simulink model "model"  (R2014a)
(part 2 of 3)

  _CN_357523602_330000_CN_87761736_330000 : powerlib/Elements/Distributed Parameters Line  Phases=3  Frequency=60  Resistance=[0.01273 0.3864]  Inductance="[0.9337e-3  4.1264e-3]"  Capacitance=[12.74e-9 7.751e-9]  Length=161.4395  x1=[0 0 0 0; 0.0001244 0 0 0; 0.0002488 0 0 0; 0.0003733 0 0 0; 0.0004977 0 0 0; 0.0006221 0 0 0]  x2=[0 0 0 0; 0.0001244 0 0 0; 0.0002488 0 0 0; 0.0003733 0 0 0; 0.0004977 0 0 0; 0.0006221 0 0 0]  x3=[0 0 0 0; 0.0001244 0 0 0; 0.0002488 0 0 0; 0.0003733 0 0 0; 0.0004977 0 0 0; 0.0006221 0 0 0]  x4=[0 0 0 0; 0.0001244 0 0 0; 0.0002488 0 0 0; 0.0003733 0 0 0; 0.0004977 0 0 0; 0.0006221 0 0 0]  x5=0  V1=ones(3,3)  V2=ones(3,3)  I1=ones(3,3)  I2=ones(3,3)  nHarmo=1  Measurements=None
  _CN_357523602_330000_CN_89072244_330000 : powerlib/Elements/Distributed Parameters Line  Phases=3  Frequency=60  Resistance=[0.01273 0.3864]  Inductance="[0.9337e-3  4.1264e-3]"  Capacitance=[12.74e-9 7.751e-9]  Length=13.8148  x1=[0 0 0 0; 0.0001244 0 0 0; 0.0002488 0 0 0; 0.0003733 0 0 0; 0.0004977 0 0 0; 0.0006221 0 0 0]  x2=[0 0 0 0; 0.0001244 0 0 0; 0.0002488 0 0 0; 0.0003733 0 0 0; 0.0004977 0 0 0; 0.0006221 0 0 0]  x3=[0 0 0 0; 0.0001244 0 0 0; 0.0002488 0 0 0; 0.0003733 0 0 0; 0.0004977 0 0 0; 0.0006221 0 0 0]  x4=[0 0 0 0; 0.0001244 0 0 0; 0.0002488 0 0 0; 0.0003733 0 0 0; 0.0004977 0 0 0; 0.0006221 0 0 0]  x5=0  V1=ones(3,3)  V2=ones(3,3)  I1=ones(3,3)  I2=ones(3,3)  nHarmo=1  Measurements=None
  _CN_42675970_110000_CN_328547675_110000 : powerlib/Elements/Distributed Parameters Line  Phases=3  Frequency=60  Resistance=[0.01273 0.3864]  Inductance="[0.9337e-3  4.1264e-3]"  Capacitance=[12.74e-9 7.751e-9]  Length=41.7952  x1=[0 0 0 0; 0.0001244 0 0 0; 0.0002488 0 0 0; 0.0003733 0 0 0; 0.0004977 0 0 0; 0.0006221 0 0 0]  x2=[0 0 0 0; 0.0001244 0 0 0; 0.0002488 0 0 0; 0.0003733 0 0 0; 0.0004977 0 0 0; 0.0006221 0 0 0]  x3=[0 0 0 0; 0.0001244 0 0 0; 0.0002488 0 0 0; 0.0003733 0 0 0; 0.0004977 0 0 0; 0.0006221 0 0 0]  x4=[0 0 0 0; 0.0001244 0 0 0; 0.0002488 0 0 0; 0.0003733 0 0 0; 0.0004977 0 0 0; 0.0006221 0 0 0]  x5=0  V1=ones(3,3)  V2=ones(3,3)  I1=ones(3,3)  I2=ones(3,3)  nHarmo=1  Measurements=None
  _CN_52300555_220000_CN_197906665_220000 : powerlib/Elements/Distributed Parameters Line  Phases=3  Frequency=60  Resistance=[0.01273 0.3864]  Inductance="[0.9337e-3  4.1264e-3]"  Capacitance=[12.74e-9 7.751e-9]  Length=149.4208  x1=[0 0 0 0; 0.0001244 0 0 0; 0.0002488 0 0 0; 0.0003733 0 0 0; 0.0004977 0 0 0; 0.0006221 0 0 0]  x2=[0 0 0 0; 0.0001244 0 0 0; 0.0002488 0 0 0; 0.0003733 0 0 0; 0.0004977 0 0 0; 0.0006221 0 0 0]  x3=[0 0 0 0; 0.0001244 0 0 0; 0.0002488 0 0 0; 0.0003733 0 0 0; 0.0004977 0 0 0; 0.0006221 0 0 0]  x4=[0 0 0 0; 0.0001244 0 0 0; 0.0002488 0 0 0; 0.0003733 0 0 0; 0.0004977 0 0 0; 0.0006221 0 0 0]  x5=0  V1=ones(3,3)  V2=ones(3,3)  I1=ones(3,3)  I2=ones(3,3)  nHarmo=1  Measurements=None
  _CN_52300555_220000_CN_315281956_220000 : powerlib/Elements/Distributed Parameters Line  Phases=3  Frequency=60  Resistance=[0.01273 0.3864]  Inductance="[0.9337e-3  4.1264e-3]"  Capacitance=[12.74e-9 7.751e-9]  Length=53.2926  x1=[0 0 0 0; 0.0001244 0 0 0; 0.0002488 0 0 0; 0.0003733 0 0 0; 0.0004977 0 0 0; 0.0006221 0 0 0]  x2=[0 0 0 0; 0.0001244 0 0 0; 0.0002488 0 0 0; 0.0003733 0 0 0; 0.0004977 0 0 0; 0.0006221 0 0 0]  x3=[0 0 0 0; 0.0001244 0 0 0; 0.0002488 0 0 0; 0.0003733 0 0 0; 0.0004977 0 0 0; 0.0006221 0 0 0]  x4=[0 0 0 0; 0.0001244 0 0 0; 0.0002488 0 0 0; 0.0003733 0 0 0; 0.0004977 0 0 0; 0.0006221 0 0 0]  x5=0  V1=ones(3,3)  V2=ones(3,3)  I1=ones(3,3)  I2=ones(3,3)  nHarmo=1  Measurements=None
  _CN_52300555_220000_CN_331268073_220000 : powerlib/Elements/Distributed Parameters Line  Phases=3  Frequency=60  Resistance=[0.01273 0.3864]  Inductance="[0.9337e-3  4.1264e-3]"  Capacitance=[12.74e-9 7.751e-9]  Length=15.583  x1=[0 0 0 0; 0.0001244 0 0 0; 0.0002488 0 0 0; 0.0003733 0 0 0; 0.0004977 0 0 0; 0.0006221 0 0 0]  x2=[0 0 0 0; 0.0001244 0 0 0; 0.0002488 0 0 0; 0.0003733 0 0 0; 0.0004977 0 0 0; 0.0006221 0 0 0]  x3=[0 0 0 0; 0.0001244 0 0 0; 0.0002488 0 0 0; 0.0003733 0 0 0; 0.0004977 0 0 0; 0.0006221 0 0 0]  x4=[0 0 0 0; 0.0001244 0 0 0; 0.0002488 0 0 0; 0.0003733 0 0 0; 0.0004977 0 0 0; 0.0006221 0 0 0]  x5=0  V1=ones(3,3)  V2=ones(3,3)  I1=ones(3,3)  I2=ones(3,3)  nHarmo=1  Measurements=None
  _CN_52300555_220000_CN_331298845_220000 : powerlib/Elements/Distributed Parameters Line  Phases=3  Frequency=60  Resistance=[0.01273 0.3864]  Inductance="[0.9337e-3  4.1264e-3]"  Capacitance=[12.74e-9 7.751e-9]  Length=186.3957  x1=[0 0 0 0; 0.0001244 0 0 0; 0.0002488 0 0 0; 0.0003733 0 0 0; 0.0004977 0 0 0; 0.0006221 0 0 0]  x2=[0 0 0 0; 0.0001244 0 0 0; 0.0002488 0 0 0; 0.0003733 0 0 0; 0.0004977 0 0 0; 0.0006221 0 0 0]  x3=[0 0 0 0; 0.0001244 0 0 0; 0.0002488 0 0 0; 0.0003733 0 0 0; 0.0004977 0 0 0; 0.0006221 0 0 0]  x4=[0 0 0 0; 0.0001244 0 0 0; 0.0002488 0 0 0; 0.0003733 0 0 0; 0.0004977 0 0 0; 0.0006221 0 0 0]  x5=0  V1=ones(3,3)  V2=ones(3,3)  I1=ones(3,3)  I2=ones(3,3)  nHarmo=1  Measurements=None
  _CN_52300555_220000_CN_96836497_220000 : powerlib/Elements/Distributed Parameters Line  Phases=3  Frequency=60  Resistance=[0.01273 0.3864]  Inductance="[0.9337e-3  4.1264e-3]"  Capacitance=[12.74e-9 7.751e-9]  Length=230.0678  x1=[0 0 0 0; 0.0001244 0 0 0; 0.0002488 0 0 0; 0.0003733 0 0 0; 0.0004977 0 0 0; 0.0006221 0 0 0]  x2=[0 0 0 0; 0.0001244 0 0 0; 0.0002488 0 0 0; 0.0003733 0 0 0; 0.0004977 0 0 0; 0.0006221 0 0 0]  x3=[0 0 0 0; 0.0001244 0 0 0; 0.0002488 0 0 0; 0.0003733 0 0 0; 0.0004977 0 0 0; 0.0006221 0 0 0]  x4=[0 0 0 0; 0.0001244 0 0 0; 0.0002488 0 0 0; 0.0003733 0 0 0; 0.0004977 0 0 0; 0.0006221 0 0 0]  x5=0  V1=ones(3,3)  V2=ones(3,3)  I1=ones(3,3)  I2=ones(3,3)  nHarmo=1  Measurements=None
  _CN_53126382_110000_CN_95829467_110000 : powerlib/Elements/Distributed Parameters Line  Phases=3  Frequency=60  Resistance=[0.01273 0.3864]  Inductance="[0.9337e-3  4.1264e-3]"  Capacitance=[12.74e-9 7.751e-9]  Length=1.7037  x1=[0 0 0 0; 0.0001244 0 0 0; 0.0002488 0 0 0; 0.0003733 0 0 0; 0.0004977 0 0 0; 0.0006221 0 0 0]  x2=[0 0 0 0; 0.0001244 0 0 0; 0.0002488 0 0 0; 0.0003733 0 0 0; 0.0004977 0 0 0; 0.0006221 0 0 0]  x3=[0 0 0 0; 0.0001244 0 0 0; 0.0002488 0 0 0; 0.0003733 0 0 0; 0.0004977 0 0 0; 0.0006221 0 0 0]  x4=[0 0 0 0; 0.0001244 0 0 0; 0.0002488 0 0 0; 0.0003733 0 0 0; 0.0004977 0 0 0; 0.0006221 0 0 0]  x5=0  V1=ones(3,3)  V2=ones(3,3)  I1=ones(3,3)  I2=ones(3,3)  nHarmo=1  Measurements=None
  _CN_55263465_110000_CN_165278014_110000 : powerlib/Elements/Distributed Parameters Line  Phases=3  Frequency=60  Resistance=[0.01273 0.3864]  Inductance="[0.9337e-3  4.1264e-3]"  Capacitance=[12.74e-9 7.751e-9]  Length=27.7089  x1=[0 0 0 0; 0.0001244 0 0 0; 0.0002488 0 0 0; 0.0003733 0 0 0; 0.0004977 0 0 0; 0.0006221 0 0 0]  x2=[0 0 0 0; 0.0001244 0 0 0; 0.0002488 0 0 0; 0.0003733 0 0 0; 0.0004977 0 0 0; 0.0006221 0 0 0]  x3=[0 0 0 0; 0.0001244 0 0 0; 0.0002488 0 0 0; 0.0003733 0 0 0; 0.0004977 0 0 0; 0.0006221 0 0 0]  x4=[0 0 0 0; 0.0001244 0 0 0; 0.0002488 0 0 0; 0.0003733 0 0 0; 0.0004977 0 0 0; 0.0006221 0 0 0]  x5=0  V1=ones(3,3)  V2=ones(3,3)  I1=ones(3,3)  I2=ones(3,3)  nHarmo=1  Measurements=None
  _CN_55263465_110000_CN_95386425_110000 : powerlib/Elements/Distributed Parameters Line  Phases=3  Frequency=60  Resistance=[0.01273 0.3864]  Inductance="[0.9337e-3  4.1264e-3]"  Capacitance=[12.74e-9 7.751e-9]  Length=7.1273  x1=[0 0 0 0; 0.0001244 0 0 0; 0.0002488 0 0 0; 0.0003733 0 0 0; 0.0004977 0 0 0; 0.0006221 0 0 0]  x2=[0 0 0 0; 0.0001244 0 0 0; 0.0002488 0 0 0; 0.0003733 0 0 0; 0.0004977 0 0 0; 0.0006221 0 0 0]  x3=[0 0 0 0; 0.0001244 0 0 0; 0.0002488 0 0 0; 0.0003733 0 0 0; 0.0004977 0 0 0; 0.0006221 0 0 0]  x4=[0 0 0 0; 0.0001244 0 0 0; 0.0002488 0 0 0; 0.0003733 0 0 0; 0.0004977 0 0 0; 0.0006221 0 0 0]  x5=0  V1=ones(3,3)  V2=ones(3,3)  I1=ones(3,3)  I2=ones(3,3)  nHarmo=1  Measurements=None
  _CN_56029959_110000_CN_142008798_110000 : powerlib/Elements/Distributed Parameters Line  Phases=3  Frequency=60  Resistance=[0.01273 0.3864]  Inductance="[0.9337e-3  4.1264e-3]"  Capacitance=[12.74e-9 7.751e-9]  Length=15.5153  x1=[0 0 0 0; 0.0001244 0 0 0; 0.0002488 0 0 0; 0.0003733 0 0 0; 0.0004977 0 0 0; 0.0006221 0 0 0]  x2=[0 0 0 0; 0.0001244 0 0 0; 0.0002488 0 0 0; 0.0003733 0 0 0; 0.0004977 0 0 0; 0.0006221 0 0 0]  x3=[0 0 0 0; 0.0001244 0 0 0; 0.0002488 0 0 0; 0.0003733 0 0 0; 0.0004977 0 0 0; 0.0006221 0 0 0]  x4=[0 0 0 0; 0.0001244 0 0 0; 0.0002488 0 0 0; 0.0003733 0 0 0; 0.0004977 0 0 0; 0.0006221 0 0 0]  x5=0  V1=ones(3,3)  V2=ones(3,3)  I1=ones(3,3)  I2=ones(3,3)  nHarmo=1  Measurements=None
  _CN_63107712_220000_CN_30831480_220000 : powerlib/Elements/Distributed Parameters Line  Phases=3  Frequency=60  Resistance=[0.01273 0.3864]  Inductance="[0.9337e-3  4.1264e-3]"  Capacitance=[12.74e-9 7.751e-9]  Length=0.67297  x1=[0 0 0 0; 0.0001244 0 0 0; 0.0002488 0 0 0; 0.0003733 0 0 0; 0.0004977 0 0 0; 0.0006221 0 0 0]  x2=[0 0 0 0; 0.0001244 0 0 0; 0.0002488 0 0 0; 0.0003733 0 0 0; 0.0004977 0 0 0; 0.0006221 0 0 0]  x3=[0 0 0 0; 0.0001244 0 0 0; 0.0002488 0 0 0; 0.0003733 0 0 0; 0.0004977 0 0 0; 0.0006221 0 0 0]  x4=[0 0 0 0; 0.0001244 0 0 0; 0.0002488 0 0 0; 0.0003733 0 0 0; 0.0004977 0 0 0; 0.0006221 0 0 0]  x5=0  V1=ones(3,3)  V2=ones(3,3)  I1=ones(3,3)  I2=ones(3,3)  nHarmo=1  Measurements=None
  _CN_74142253_110000_CN_104487370_110000 : powerlib/Elements/Distributed Parameters Line  Phases=3  Frequency=60  Resistance=[0.01273 0.3864]  Inductance="[0.9337e-3  4.1264e-3]"  Capacitance=[12.74e-9 7.751e-9]  Length=2.4161  x1=[0 0 0 0; 0.0001244 0 0 0; 0.0002488 0 0 0; 0.0003733 0 0 0; 0.0004977 0 0 0; 0.0006221 0 0 0]  x2=[0 0 0 0; 0.0001244 0 0 0; 0.0002488 0 0 0; 0.0003733 0 0 0; 0.0004977 0 0 0; 0.0006221 0 0 0]  x3=[0 0 0 0; 0.0001244 0 0 0; 0.0002488 0 0 0; 0.0003733 0 0 0; 0.0004977 0 0 0; 0.0006221 0 0 0]  x4=[0 0 0 0; 0.0001244 0 0 0; 0.0002488 0 0 0; 0.0003733 0 0 0; 0.0004977 0 0 0; 0.0006221 0 0 0]  x5=0  V1=ones(3,3)  V2=ones(3,3)  I1=ones(3,3)  I2=ones(3,3)  nHarmo=1  Measurements=None
  _CN_75305342_110000_CN_46035010_110000 : powerlib/Elements/Distributed Parameters Line  Phases=3  Frequency=60  Resistance=[0.01273 0.3864]  Inductance="[0.9337e-3  4.1264e-3]"  Capacitance=[12.74e-9 7.751e-9]  Length=8.5727  x1=[0 0 0 0; 0.0001244 0 0 0; 0.0002488 0 0 0; 0.0003733 0 0 0; 0.0004977 0 0 0; 0.0006221 0 0 0]  x2=[0 0 0 0; 0.0001244 0 0 0; 0.0002488 0 0 0; 0.0003733 0 0 0; 0.0004977 0 0 0; 0.0006221 0 0 0]  x3=[0 0 0 0; 0.0001244 0 0 0; 0.0002488 0 0 0; 0.0003733 0 0 0; 0.0004977 0 0 0; 0.0006221 0 0 0]  x4=[0 0 0 0; 0.0001244 0 0 0; 0.0002488 0 0 0; 0.0003733 0 0 0; 0.0004977 0 0 0; 0.0006221 0 0 0]  x5=0  V1=ones(3,3)  V2=ones(3,3)  I1=ones(3,3)  I2=ones(3,3)  nHarmo=1  Measurements=None
  _CN_87430145_220000_CN_105528914_220000 : powerlib/Elements/Distributed Parameters Line  Phases=3  Frequency=60  Resistance=[0.01273 0.3864]  Inductance="[0.9337e-3  4.1264e-3]"  Capacitance=[12.74e-9 7.751e-9]  Length=102.2998  x1=[0 0 0 0; 0.0001244 0 0 0; 0.0002488 0 0 0; 0.0003733 0 0 0; 0.0004977 0 0 0; 0.0006221 0 0 0]  x2=[0 0 0 0; 0.0001244 0 0 0; 0.0002488 0 0 0; 0.0003733 0 0 0; 0.0004977 0 0 0; 0.0006221 0 0 0]  x3=[0 0 0 0; 0.0001244 0 0 0; 0.0002488 0 0 0; 0.0003733 0 0 0; 0.0004977 0 0 0; 0.0006221 0 0 0]  x4=[0 0 0 0; 0.0001244 0 0 0; 0.0002488 0 0 0; 0.0003733 0 0 0; 0.0004977 0 0 0; 0.0006221 0 0 0]  x5=0  V1=ones(3,3)  V2=ones(3,3)  I1=ones(3,3)  I2=ones(3,3)  nHarmo=1  Measurements=None
  _CN_87430145_220000_CN_106941567_220000 : powerlib/Elements/Distributed Parameters Line  Phases=3  Frequency=60  Resistance=[0.01273 0.3864]  Inductance="[0.9337e-3  4.1264e-3]"  Capacitance=[12.74e-9 7.751e-9]  Length=3.6587  x1=[0 0 0 0; 0.0001244 0 0 0; 0.0002488 0 0 0; 0.0003733 0 0 0; 0.0004977 0 0 0; 0.0006221 0 0 0]  x2=[0 0 0 0; 0.0001244 0 0 0; 0.0002488 0 0 0; 0.0003733 0 0 0; 0.0004977 0 0 0; 0.0006221 0 0 0]  x3=[0 0 0 0; 0.0001244 0 0 0; 0.0002488 0 0 0; 0.0003733 0 0 0; 0.0004977 0 0 0; 0.0006221 0 0 0]  x4=[0 0 0 0; 0.0001244 0 0 0; 0.0002488 0 0 0; 0.0003733 0 0 0; 0.0004977 0 0 0; 0.0006221 0 0 0]  x5=0  V1=ones(3,3)  V2=ones(3,3)  I1=ones(3,3)  I2=ones(3,3)  nHarmo=1  Measurements=None
  _CN_87430145_220000_CN_88433653_220000 : powerlib/Elements/Distributed Parameters Line  Phases=3  Frequency=60  Resistance=[0.01273 0.3864]  Inductance="[0.9337e-3  4.1264e-3]"  Capacitance=[12.74e-9 7.751e-9]  Length=266.7352  x1=[0 0 0 0; 0.0001244 0 0 0; 0.0002488 0 0 0; 0.0003733 0 0 0; 0.0004977 0 0 0; 0.0006221 0 0 0]  x2=[0 0 0 0; 0.0001244 0 0 0; 0.0002488 0 0 0; 0.0003733 0 0 0; 0.0004977 0 0 0; 0.0006221 0 0 0]  x3=[0 0 0 0; 0.0001244 0 0 0; 0.0002488 0 0 0; 0.0003733 0 0 0; 0.0004977 0 0 0; 0.0006221 0 0 0]  x4=[0 0 0 0; 0.0001244 0 0 0; 0.0002488 0 0 0; 0.0003733 0 0 0; 0.0004977 0 0 0; 0.0006221 0 0 0]  x5=0  V1=ones(3,3)  V2=ones(3,3)  I1=ones(3,3)  I2=ones(3,3)  nHarmo=1  Measurements=None
  _CN_87761736_330000_CN_161733477_330000 : powerlib/Elements/Distributed Parameters Line  Phases=3  Frequency=60  Resistance=[0.01273 0.3864]  Inductance="[0.9337e-3  4.1264e-3]"  Capacitance=[12.74e-9 7.751e-9]  Length=34.7035  x1=[0 0 0 0; 0.0001244 0 0 0; 0.0002488 0 0 0; 0.0003733 0 0 0; 0.0004977 0 0 0; 0.0006221 0 0 0]  x2=[0 0 0 0; 0.0001244 0 0 0; 0.0002488 0 0 0; 0.0003733 0 0 0; 0.0004977 0 0 0; 0.0006221 0 0 0]  x3=[0 0 0 0; 0.0001244 0 0 0; 0.0002488 0 0 0; 0.0003733 0 0 0; 0.0004977 0 0 0; 0.0006221 0 0 0]  x4=[0 0 0 0; 0.0001244 0 0 0; 0.0002488 0 0 0; 0.0003733 0 0 0; 0.0004977 0 0 0; 0.0006221 0 0 0]  x5=0  V1=ones(3,3)  V2=ones(3,3)  I1=ones(3,3)  I2=ones(3,3)  nHarmo=1  Measurements=None
  _CN_87761736_330000_CN_34682059_330000 : powerlib/Elements/Distributed Parameters Line  Phases=3  Frequency=60  Resistance=[0.01273 0.3864]  Inductance="[0.9337e-3  4.1264e-3]"  Capacitance=[12.74e-9 7.751e-9]  Length=172.6309  x1=[0 0 0 0; 0.0001244 0 0 0; 0.0002488 0 0 0; 0.0003733 0 0 0; 0.0004977 0 0 0; 0.0006221 0 0 0]  x2=[0 0 0 0; 0.0001244 0 0 0; 0.0002488 0 0 0; 0.0003733 0 0 0; 0.0004977 0 0 0; 0.0006221 0 0 0]  x3=[0 0 0 0; 0.0001244 0 0 0; 0.0002488 0 0 0; 0.0003733 0 0 0; 0.0004977 0 0 0; 0.0006221 0 0 0]  x4=[0 0 0 0; 0.0001244 0 0 0; 0.0002488 0 0 0; 0.0003733 0 0 0; 0.0004977 0 0 0; 0.0006221 0 0 0]  x5=0  V1=ones(3,3)  V2=ones(3,3)  I1=ones(3,3)  I2=ones(3,3)  nHarmo=1  Measurements=None
  _CN_97385278_110000_CN_302320627_110000 : powerlib/Elements/Distributed Parameters Line  Phases=3  Frequency=60  Resistance=[0.01273 0.3864]  Inductance="[0.9337e-3  4.1264e-3]"  Capacitance=[12.74e-9 7.751e-9]  Length=14.0275  x1=[0 0 0 0; 0.0001244 0 0 0; 0.0002488 0 0 0; 0.0003733 0 0 0; 0.0004977 0 0 0; 0.0006221 0 0 0]  x2=[0 0 0 0; 0.0001244 0 0 0; 0.0002488 0 0 0; 0.0003733 0 0 0; 0.0004977 0 0 0; 0.0006221 0 0 0]  x3=[0 0 0 0; 0.0001244 0 0 0; 0.0002488 0 0 0; 0.0003733 0 0 0; 0.0004977 0 0 0; 0.0006221 0 0 0]  x4=[0 0 0 0; 0.0001244 0 0 0; 0.0002488 0 0 0; 0.0003733 0 0 0; 0.0004977 0 0 0; 0.0006221 0 0 0]  x5=0  V1=ones(3,3)  V2=ones(3,3)  I1=ones(3,3)  I2=ones(3,3)  nHarmo=1  Measurements=None
  bus1 : powerlib/Measurements/Load Flow Bus  LConnTagsString=a  ID=bus1  Vbase=110000  Vref=1  Vangle=0  VLF=1  angleLF=0
      settings: AttributesFormatString=|
      | %<ID>
      | %<Vbase>V
      | %<VLF>pu
      | %<angleLF>deg.
      | %<Name>
  bus10 : powerlib/Measurements/Load Flow Bus  LConnTagsString=a  ID=bus10  Vbase=110000  Vref=1  Vangle=0  VLF=1  angleLF=0
      settings: AttributesFormatString=|
      | %<ID>
      | %<Vbase>V
      | %<VLF>pu
      | %<angleLF>deg.
      | %<Name>
  bus100 : powerlib/Measurements/Load Flow Bus  LConnTagsString=a  ID=bus100  Vbase=110000  Vref=1  Vangle=0  VLF=1  angleLF=0
      settings: AttributesFormatString=|
      | %<ID>
      | %<Vbase>V
      | %<VLF>pu
      | %<angleLF>deg.
      | %<Name>
  bus101 : powerlib/Measurements/Load Flow Bus  LConnTagsString=a  ID=bus101  Vbase=110000  Vref=1  Vangle=0  VLF=1  angleLF=0
      settings: AttributesFormatString=|
      | %<ID>
      | %<Vbase>V
      | %<VLF>pu
      | %<angleLF>deg.
      | %<Name>
  bus102 : powerlib/Measurements/Load Flow Bus  LConnTagsString=a  ID=bus102  Vbase=110000  Vref=1  Vangle=0  VLF=1  angleLF=0
      settings: AttributesFormatString=|
      | %<ID>
      | %<Vbase>V
      | %<VLF>pu
      | %<angleLF>deg.
      | %<Name>
  bus103 : powerlib/Measurements/Load Flow Bus  LConnTagsString=a  ID=bus103  Vbase=220000  Vref=1  Vangle=0  VLF=1  angleLF=0
      settings: AttributesFormatString=|
      | %<ID>
      | %<Vbase>V
      | %<VLF>pu
      | %<angleLF>deg.
      | %<Name>
  bus104 : powerlib/Measurements/Load Flow Bus  LConnTagsString=a  ID=bus104  Vbase=220000  Vref=1  Vangle=0  VLF=1  angleLF=0
      settings: AttributesFormatString=|
      | %<ID>
      | %<Vbase>V
      | %<VLF>pu
      | %<angleLF>deg.
      | %<Name>
  bus105 : powerlib/Measurements/Load Flow Bus  LConnTagsString=a  ID=bus105  Vbase=220000  Vref=1  Vangle=0  VLF=1  angleLF=0
      settings: AttributesFormatString=|
      | %<ID>
      | %<Vbase>V
      | %<VLF>pu
      | %<angleLF>deg.
      | %<Name>
  bus106 : powerlib/Measurements/Load Flow Bus  LConnTagsString=a  ID=bus106  Vbase=220000  Vref=1  Vangle=0  VLF=1  angleLF=0
      settings: AttributesFormatString=|
      | %<ID>
      | %<Vbase>V
      | %<VLF>pu
      | %<angleLF>deg.
      | %<Name>
  bus107 : powerlib/Measurements/Load Flow Bus  LConnTagsString=a  ID=bus107  Vbase=220000  Vref=1  Vangle=0  VLF=1  angleLF=0
      settings: AttributesFormatString=|
      | %<ID>
      | %<Vbase>V
      | %<VLF>pu
      | %<angleLF>deg.
      | %<Name>
  bus108 : powerlib/Measurements/Load Flow Bus  LConnTagsString=a  ID=bus108  Vbase=220000  Vref=1  Vangle=0  VLF=1  angleLF=0
      settings: AttributesFormatString=|
      | %<ID>
      | %<Vbase>V
      | %<VLF>pu
      | %<angleLF>deg.
      | %<Name>
  bus109 : powerlib/Measurements/Load Flow Bus  LConnTagsString=a  ID=bus109  Vbase=220000  Vref=1  Vangle=0  VLF=1  angleLF=0
      settings: AttributesFormatString=|
      | %<ID>
      | %<Vbase>V
      | %<VLF>pu
      | %<angleLF>deg.
      | %<Name>
  bus11 : powerlib/Measurements/Load Flow Bus  LConnTagsString=a  ID=bus11  Vbase=110000  Vref=1  Vangle=0  VLF=1  angleLF=0
      settings: AttributesFormatString=|
      | %<ID>
      | %<Vbase>V
      | %<VLF>pu
      | %<angleLF>deg.
      | %<Name>
  bus110 : powerlib/Measurements/Load Flow Bus  LConnTagsString=a  ID=bus110  Vbase=220000  Vref=1  Vangle=0  VLF=1  angleLF=0
      settings: AttributesFormatString=|
      | %<ID>
      | %<Vbase>V
      | %<VLF>pu
      | %<angleLF>deg.
      | %<Name>
  bus111 : powerlib/Measurements/Load Flow Bus  LConnTagsString=a  ID=bus111  Vbase=220000  Vref=1  Vangle=0  VLF=1  angleLF=0
      settings: AttributesFormatString=|
      | %<ID>
      | %<Vbase>V
      | %<VLF>pu
      | %<angleLF>deg.
      | %<Name>
  bus112 : powerlib/Measurements/Load Flow Bus  LConnTagsString=a  ID=bus112  Vbase=220000  Vref=1  Vangle=0  VLF=1  angleLF=0
      settings: AttributesFormatString=|
      | %<ID>
      | %<Vbase>V
      | %<VLF>pu
      | %<angleLF>deg.
      | %<Name>
  bus113 : powerlib/Measurements/Load Flow Bus  LConnTagsString=a  ID=bus113  Vbase=220000  Vref=1  Vangle=0  VLF=1  angleLF=0
      settings: AttributesFormatString=|
      | %<ID>
      | %<Vbase>V
      | %<VLF>pu
      | %<angleLF>deg.
      | %<Name>
  bus114 : powerlib/Measurements/Load Flow Bus  LConnTagsString=a  ID=bus114  Vbase=220000  Vref=1  Vangle=0  VLF=1  angleLF=0
      settings: AttributesFormatString=|
      | %<ID>
      | %<Vbase>V
      | %<VLF>pu
      | %<angleLF>deg.
      | %<Name>
  bus115 : powerlib/Measurements/Load Flow Bus  LConnTagsString=a  ID=bus115  Vbase=220000  Vref=1  Vangle=0  VLF=1  angleLF=0
      settings: AttributesFormatString=|
      | %<ID>
      | %<Vbase>V
      | %<VLF>pu
      | %<angleLF>deg.
      | %<Name>
  bus116 : powerlib/Measurements/Load Flow Bus  LConnTagsString=a  ID=bus116  Vbase=220000  Vref=1  Vangle=0  VLF=1  angleLF=0
      settings: AttributesFormatString=|
      | %<ID>
      | %<Vbase>V
      | %<VLF>pu
      | %<angleLF>deg.
      | %<Name>
  bus117 : powerlib/Measurements/Load Flow Bus  LConnTagsString=a  ID=bus117  Vbase=220000  Vref=1  Vangle=0  VLF=1  angleLF=0
      settings: AttributesFormatString=|
      | %<ID>
      | %<Vbase>V
      | %<VLF>pu
      | %<angleLF>deg.
      | %<Name>
  bus118 : powerlib/Measurements/Load Flow Bus  LConnTagsString=a  ID=bus118  Vbase=220000  Vref=1  Vangle=0  VLF=1  angleLF=0
      settings: AttributesFormatString=|
      | %<ID>
      | %<Vbase>V
      | %<VLF>pu
      | %<angleLF>deg.
      | %<Name>
  bus119 : powerlib/Measurements/Load Flow Bus  LConnTagsString=a  ID=bus119  Vbase=220000  Vref=1  Vangle=0  VLF=1  angleLF=0
      settings: AttributesFormatString=|
      | %<ID>
      | %<Vbase>V
      | %<VLF>pu
      | %<angleLF>deg.
      | %<Name>
  bus12 : powerlib/Measurements/Load Flow Bus  LConnTagsString=a  ID=bus12  Vbase=110000  Vref=1  Vangle=0  VLF=1  angleLF=0
      settings: AttributesFormatString=|
      | %<ID>
      | %<Vbase>V
      | %<VLF>pu
      | %<angleLF>deg.
      | %<Name>
  bus120 : powerlib/Measurements/Load Flow Bus  LConnTagsString=a  ID=bus120  Vbase=220000  Vref=1  Vangle=0  VLF=1  angleLF=0
      settings: AttributesFormatString=|
      | %<ID>
      | %<Vbase>V
      | %<VLF>pu
      | %<angleLF>deg.
      | %<Name>
  bus121 : powerlib/Measurements/Load Flow Bus  LConnTagsString=a  ID=bus121  Vbase=220000  Vref=1  Vangle=0  VLF=1  angleLF=0
      settings: AttributesFormatString=|
      | %<ID>
      | %<Vbase>V
      | %<VLF>pu
      | %<angleLF>deg.
      | %<Name>
  bus122 : powerlib/Measurements/Load Flow Bus  LConnTagsString=a  ID=bus122  Vbase=220000  Vref=1  Vangle=0  VLF=1  angleLF=0
      settings: AttributesFormatString=|
      | %<ID>
      | %<Vbase>V
      | %<VLF>pu
      | %<angleLF>deg.
      | %<Name>
  bus123 : powerlib/Measurements/Load Flow Bus  LConnTagsString=a  ID=bus123  Vbase=220000  Vref=1  Vangle=0  VLF=1  angleLF=0
      settings: AttributesFormatString=|
      | %<ID>
      | %<Vbase>V
      | %<VLF>pu
      | %<angleLF>deg.
      | %<Name>
  bus124 : powerlib/Measurements/Load Flow Bus  LConnTagsString=a  ID=bus124  Vbase=220000  Vref=1  Vangle=0  VLF=1  angleLF=0
      settings: AttributesFormatString=|
      | %<ID>
      | %<Vbase>V
      | %<VLF>pu
      | %<angleLF>deg.
      | %<Name>
  bus125 : powerlib/Measurements/Load Flow Bus  LConnTagsString=a  ID=bus125  Vbase=220000  Vref=1  Vangle=0  VLF=1  angleLF=0
      settings: AttributesFormatString=|
      | %<ID>
      | %<Vbase>V
      | %<VLF>pu
      | %<angleLF>deg.
      | %<Name>
  bus126 : powerlib/Measurements/Load Flow Bus  LConnTagsString=a  ID=bus126  Vbase=220000  Vref=1  Vangle=0  VLF=1  angleLF=0
      settings: AttributesFormatString=|
      | %<ID>
      | %<Vbase>V
      | %<VLF>pu
      | %<angleLF>deg.
      | %<Name>
  bus127 : powerlib/Measurements/Load Flow Bus  LConnTagsString=a  ID=bus127  Vbase=220000  Vref=1  Vangle=0  VLF=1  angleLF=0
      settings: AttributesFormatString=|
      | %<ID>
      | %<Vbase>V
      | %<VLF>pu
      | %<angleLF>deg.
      | %<Name>
  bus128 : powerlib/Measurements/Load Flow Bus  LConnTagsString=a  ID=bus128  Vbase=220000  Vref=1  Vangle=0  VLF=1  angleLF=0
      settings: AttributesFormatString=|
      | %<ID>
      | %<Vbase>V
      | %<VLF>pu
      | %<angleLF>deg.
      | %<Name>
  bus129 : powerlib/Measurements/Load Flow Bus  LConnTagsString=a  ID=bus129  Vbase=220000  Vref=1  Vangle=0  VLF=1  angleLF=0
      settings: AttributesFormatString=|
      | %<ID>
      | %<Vbase>V
      | %<VLF>pu
      | %<angleLF>deg.
      | %<Name>
  bus13 : powerlib/Measurements/Load Flow Bus  LConnTagsString=a  ID=bus13  Vbase=110000  Vref=1  Vangle=0  VLF=1  angleLF=0
      settings: AttributesFormatString=|
      | %<ID>
      | %<Vbase>V
      | %<VLF>pu
      | %<angleLF>deg.
      | %<Name>
  bus130 : powerlib/Measurements/Load Flow Bus  LConnTagsString=a  ID=bus130  Vbase=220000  Vref=1  Vangle=0  VLF=1  angleLF=0
      settings: AttributesFormatString=|
      | %<ID>
      | %<Vbase>V
      | %<VLF>pu
      | %<angleLF>deg.
      | %<Name>
  bus131 : powerlib/Measurements/Load Flow Bus  LConnTagsString=a  ID=bus131  Vbase=220000  Vref=1  Vangle=0  VLF=1  angleLF=0
      settings: AttributesFormatString=|
      | %<ID>
      | %<Vbase>V
      | %<VLF>pu
      | %<angleLF>deg.
      | %<Name>
  bus132 : powerlib/Measurements/Load Flow Bus  LConnTagsString=a  ID=bus132  Vbase=220000  Vref=1  Vangle=0  VLF=1  angleLF=0
      settings: AttributesFormatString=|
      | %<ID>
      | %<Vbase>V
      | %<VLF>pu
      | %<angleLF>deg.
      | %<Name>
  bus133 : powerlib/Measurements/Load Flow Bus  LConnTagsString=a  ID=bus133  Vbase=220000  Vref=1  Vangle=0  VLF=1  angleLF=0
      settings: AttributesFormatString=|
      | %<ID>
      | %<Vbase>V
      | %<VLF>pu
      | %<angleLF>deg.
      | %<Name>
  bus134 : powerlib/Measurements/Load Flow Bus  LConnTagsString=a  ID=bus134  Vbase=330000  Vref=1  Vangle=0  VLF=1  angleLF=0
      settings: AttributesFormatString=|
      | %<ID>
      | %<Vbase>V
      | %<VLF>pu
      | %<angleLF>deg.
      | %<Name>
  bus135 : powerlib/Measurements/Load Flow Bus  LConnTagsString=a  ID=bus135  Vbase=330000  Vref=1  Vangle=0  VLF=1  angleLF=0
      settings: AttributesFormatString=|
      | %<ID>
      | %<Vbase>V
      | %<VLF>pu
      | %<angleLF>deg.
      | %<Name>
  bus136 : powerlib/Measurements/Load Flow Bus  LConnTagsString=a  ID=bus136  Vbase=330000  Vref=1  Vangle=0  VLF=1  angleLF=0
      settings: AttributesFormatString=|
      | %<ID>
      | %<Vbase>V
      | %<VLF>pu
      | %<angleLF>deg.
      | %<Name>
  bus137 : powerlib/Measurements/Load Flow Bus  LConnTagsString=a  ID=bus137  Vbase=330000  Vref=1  Vangle=0  VLF=1  angleLF=0
      settings: AttributesFormatString=|
      | %<ID>
      | %<Vbase>V
      | %<VLF>pu
      | %<angleLF>deg.
      | %<Name>
  bus138 : powerlib/Measurements/Load Flow Bus  LConnTagsString=a  ID=bus138  Vbase=330000  Vref=1  Vangle=0  VLF=1  angleLF=0
      settings: AttributesFormatString=|
      | %<ID>
      | %<Vbase>V
      | %<VLF>pu
      | %<angleLF>deg.
      | %<Name>
  bus139 : powerlib/Measurements/Load Flow Bus  LConnTagsString=a  ID=bus139  Vbase=330000  Vref=1  Vangle=0  VLF=1  angleLF=0
      settings: AttributesFormatString=|
      | %<ID>
      | %<Vbase>V
      | %<VLF>pu
      | %<angleLF>deg.
      | %<Name>
  bus14 : powerlib/Measurements/Load Flow Bus  LConnTagsString=a  ID=bus14  Vbase=110000  Vref=1  Vangle=0  VLF=1  angleLF=0
      settings: AttributesFormatString=|
      | %<ID>
      | %<Vbase>V
      | %<VLF>pu
      | %<angleLF>deg.
      | %<Name>
  bus140 : powerlib/Measurements/Load Flow Bus  LConnTagsString=a  ID=bus140  Vbase=330000  Vref=1  Vangle=0  VLF=1  angleLF=0
      settings: AttributesFormatString=|
      | %<ID>
      | %<Vbase>V
      | %<VLF>pu
      | %<angleLF>deg.
      | %<Name>
  bus141 : powerlib/Measurements/Load Flow Bus  LConnTagsString=a  ID=bus141  Vbase=330000  Vref=1  Vangle=0  VLF=1  angleLF=0
      settings: AttributesFormatString=|
      | %<ID>
      | %<Vbase>V
      | %<VLF>pu
      | %<angleLF>deg.
      | %<Name>
  bus142 : powerlib/Measurements/Load Flow Bus  LConnTagsString=a  ID=bus142  Vbase=330000  Vref=1  Vangle=0  VLF=1  angleLF=0
      settings: AttributesFormatString=|
      | %<ID>
      | %<Vbase>V
      | %<VLF>pu
      | %<angleLF>deg.
      | %<Name>
  bus143 : powerlib/Measurements/Load Flow Bus  LConnTagsString=a  ID=bus143  Vbase=330000  Vref=1  Vangle=0  VLF=1  angleLF=0
      settings: AttributesFormatString=|
      | %<ID>
      | %<Vbase>V
      | %<VLF>pu
      | %<angleLF>deg.
      | %<Name>
  bus144 : powerlib/Measurements/Load Flow Bus  LConnTagsString=a  ID=bus144  Vbase=330000  Vref=1  Vangle=0  VLF=1  angleLF=0
      settings: AttributesFormatString=|
      | %<ID>
      | %<Vbase>V
      | %<VLF>pu
      | %<angleLF>deg.
      | %<Name>
  bus145 : powerlib/Measurements/Load Flow Bus  LConnTagsString=a  ID=bus145  Vbase=330000  Vref=1  Vangle=0  VLF=1  angleLF=0
      settings: AttributesFormatString=|
      | %<ID>
      | %<Vbase>V
      | %<VLF>pu
      | %<angleLF>deg.
      | %<Name>
  bus146 : powerlib/Measurements/Load Flow Bus  LConnTagsString=a  ID=bus146  Vbase=330000  Vref=1  Vangle=0  VLF=1  angleLF=0
      settings: AttributesFormatString=|
      | %<ID>
      | %<Vbase>V
      | %<VLF>pu
      | %<angleLF>deg.
      | %<Name>
  bus147 : powerlib/Measurements/Load Flow Bus  LConnTagsString=a  ID=bus147  Vbase=330000  Vref=1  Vangle=0  VLF=1  angleLF=0
      settings: AttributesFormatString=|
      | %<ID>
      | %<Vbase>V
      | %<VLF>pu
      | %<angleLF>deg.
      | %<Name>
  bus148 : powerlib/Measurements/Load Flow Bus  LConnTagsString=a  ID=bus148  Vbase=330000  Vref=1  Vangle=0  VLF=1  angleLF=0
      settings: AttributesFormatString=|
      | %<ID>
      | %<Vbase>V
      | %<VLF>pu
      | %<angleLF>deg.
      | %<Name>
  bus149 : powerlib/Measurements/Load Flow Bus  LConnTagsString=a  ID=bus149  Vbase=330000  Vref=1  Vangle=0  VLF=1  angleLF=0
      settings: AttributesFormatString=|
      | %<ID>
      | %<Vbase>V
      | %<VLF>pu
      | %<angleLF>deg.
      | %<Name>
  bus15 : powerlib/Measurements/Load Flow Bus  LConnTagsString=a  ID=bus15  Vbase=110000  Vref=1  Vangle=0  VLF=1  angleLF=0
      settings: AttributesFormatString=|
      | %<ID>
      | %<Vbase>V
      | %<VLF>pu
      | %<angleLF>deg.
      | %<Name>
  bus150 : powerlib/Measurements/Load Flow Bus  LConnTagsString=a  ID=bus150  Vbase=330000  Vref=1  Vangle=0  VLF=1  angleLF=0
      settings: AttributesFormatString=|
      | %<ID>
      | %<Vbase>V
      | %<VLF>pu
      | %<angleLF>deg.
      | %<Name>
  bus151 : powerlib/Measurements/Load Flow Bus  LConnTagsString=a  ID=bus151  Vbase=330000  Vref=1  Vangle=0  VLF=1  angleLF=0
      settings: AttributesFormatString=|
      | %<ID>
      | %<Vbase>V
      | %<VLF>pu
      | %<angleLF>deg.
      | %<Name>
  bus152 : powerlib/Measurements/Load Flow Bus  LConnTagsString=a  ID=bus152  Vbase=330000  Vref=1  Vangle=0  VLF=1  angleLF=0
      settings: AttributesFormatString=|
      | %<ID>
      | %<Vbase>V
      | %<VLF>pu
      | %<angleLF>deg.
      | %<Name>
  bus153 : powerlib/Measurements/Load Flow Bus  LConnTagsString=a  ID=bus153  Vbase=330000  Vref=1  Vangle=0  VLF=1  angleLF=0
      settings: AttributesFormatString=|
      | %<ID>
      | %<Vbase>V
      | %<VLF>pu
      | %<angleLF>deg.
      | %<Name>
  bus154 : powerlib/Measurements/Load Flow Bus  LConnTagsString=a  ID=bus154  Vbase=330000  Vref=1  Vangle=0  VLF=1  angleLF=0
      settings: AttributesFormatString=|
      | %<ID>
      | %<Vbase>V
      | %<VLF>pu
      | %<angleLF>deg.
      | %<Name>
  bus155 : powerlib/Measurements/Load Flow Bus  LConnTagsString=a  ID=bus155  Vbase=330000  Vref=1  Vangle=0  VLF=1  angleLF=0
      settings: AttributesFormatString=|
      | %<ID>
      | %<Vbase>V
      | %<VLF>pu
      | %<angleLF>deg.
      | %<Name>
  bus156 : powerlib/Measurements/Load Flow Bus  LConnTagsString=a  ID=bus156  Vbase=330000  Vref=1  Vangle=0  VLF=1  angleLF=0
      settings: AttributesFormatString=|
      | %<ID>
      | %<Vbase>V
      | %<VLF>pu
      | %<angleLF>deg.
      | %<Name>
  bus157 : powerlib/Measurements/Load Flow Bus  LConnTagsString=a  ID=bus157  Vbase=330000  Vref=1  Vangle=0  VLF=1  angleLF=0
      settings: AttributesFormatString=|
      | %<ID>
      | %<Vbase>V
      | %<VLF>pu
      | %<angleLF>deg.
      | %<Name>
  bus158 : powerlib/Measurements/Load Flow Bus  LConnTagsString=a  ID=bus158  Vbase=330000  Vref=1  Vangle=0  VLF=1  angleLF=0
      settings: AttributesFormatString=|
      | %<ID>
      | %<Vbase>V
      | %<VLF>pu
      | %<angleLF>deg.
      | %<Name>
  bus159 : powerlib/Measurements/Load Flow Bus  LConnTagsString=a  ID=bus159  Vbase=110000  Vref=1  Vangle=0  VLF=1  angleLF=0
      settings: AttributesFormatString=|
      | %<ID>
      | %<Vbase>V
      | %<VLF>pu
      | %<angleLF>deg.
      | %<Name>
  bus16 : powerlib/Measurements/Load Flow Bus  LConnTagsString=a  ID=bus16  Vbase=110000  Vref=1  Vangle=0  VLF=1  angleLF=0
      settings: AttributesFormatString=|
      | %<ID>
      | %<Vbase>V
      | %<VLF>pu
      | %<angleLF>deg.
      | %<Name>
  bus160 : powerlib/Measurements/Load Flow Bus  LConnTagsString=a  ID=bus160  Vbase=110000  Vref=1  Vangle=0  VLF=1  angleLF=0
      settings: AttributesFormatString=|
      | %<ID>
      | %<Vbase>V
      | %<VLF>pu
      | %<angleLF>deg.
      | %<Name>
  bus161 : powerlib/Measurements/Load Flow Bus  LConnTagsString=a  ID=bus161  Vbase=110000  Vref=1  Vangle=0  VLF=1  angleLF=0
      settings: AttributesFormatString=|
      | %<ID>
      | %<Vbase>V
      | %<VLF>pu
      | %<angleLF>deg.
      | %<Name>
  bus162 : powerlib/Measurements/Load Flow Bus  LConnTagsString=a  ID=bus162  Vbase=110000  Vref=1  Vangle=0  VLF=1  angleLF=0
      settings: AttributesFormatString=|
      | %<ID>
      | %<Vbase>V
      | %<VLF>pu
      | %<angleLF>deg.
      | %<Name>
  bus163 : powerlib/Measurements/Load Flow Bus  LConnTagsString=a  ID=bus163  Vbase=110000  Vref=1  Vangle=0  VLF=1  angleLF=0
      settings: AttributesFormatString=|
      | %<ID>
      | %<Vbase>V
      | %<VLF>pu
      | %<angleLF>deg.
      | %<Name>
  bus164 : powerlib/Measurements/Load Flow Bus  LConnTagsString=a  ID=bus164  Vbase=110000  Vref=1  Vangle=0  VLF=1  angleLF=0
      settings: AttributesFormatString=|
      | %<ID>
      | %<Vbase>V
      | %<VLF>pu
      | %<angleLF>deg.
      | %<Name>
  bus165 : powerlib/Measurements/Load Flow Bus  LConnTagsString=a  ID=bus165  Vbase=110000  Vref=1  Vangle=0  VLF=1  angleLF=0
      settings: AttributesFormatString=|
      | %<ID>
      | %<Vbase>V
      | %<VLF>pu
      | %<angleLF>deg.
      | %<Name>
  bus166 : powerlib/Measurements/Load Flow Bus  LConnTagsString=a  ID=bus166  Vbase=110000  Vref=1  Vangle=0  VLF=1  angleLF=0
      settings: AttributesFormatString=|
      | %<ID>
      | %<Vbase>V
      | %<VLF>pu
      | %<angleLF>deg.
      | %<Name>
  bus167 : powerlib/Measurements/Load Flow Bus  LConnTagsString=a  ID=bus167  Vbase=110000  Vref=1  Vangle=0  VLF=1  angleLF=0
      settings: AttributesFormatString=|
      | %<ID>
      | %<Vbase>V
      | %<VLF>pu
      | %<angleLF>deg.
      | %<Name>
  bus168 : powerlib/Measurements/Load Flow Bus  LConnTagsString=a  ID=bus168  Vbase=110000  Vref=1  Vangle=0  VLF=1  angleLF=0
      settings: AttributesFormatString=|
      | %<ID>
      | %<Vbase>V
      | %<VLF>pu
      | %<angleLF>deg.
      | %<Name>
  bus169 : powerlib/Measurements/Load Flow Bus  LConnTagsString=a  ID=bus169  Vbase=110000  Vref=1  Vangle=0  VLF=1  angleLF=0
      settings: AttributesFormatString=|
      | %<ID>
      | %<Vbase>V
      | %<VLF>pu
      | %<angleLF>deg.
      | %<Name>
  bus17 : powerlib/Measurements/Load Flow Bus  LConnTagsString=a  ID=bus17  Vbase=110000  Vref=1  Vangle=0  VLF=1  angleLF=0
      settings: AttributesFormatString=|
      | %<ID>
      | %<Vbase>V
      | %<VLF>pu
      | %<angleLF>deg.
      | %<Name>
  bus170 : powerlib/Measurements/Load Flow Bus  LConnTagsString=a  ID=bus170  Vbase=110000  Vref=1  Vangle=0  VLF=1  angleLF=0
      settings: AttributesFormatString=|
      | %<ID>
      | %<Vbase>V
      | %<VLF>pu
      | %<angleLF>deg.
      | %<Name>
  bus171 : powerlib/Measurements/Load Flow Bus  LConnTagsString=a  ID=bus171  Vbase=110000  Vref=1  Vangle=0  VLF=1  angleLF=0
      settings: AttributesFormatString=|
      | %<ID>
      | %<Vbase>V
      | %<VLF>pu
      | %<angleLF>deg.
      | %<Name>
  bus172 : powerlib/Measurements/Load Flow Bus  LConnTagsString=a  ID=bus172  Vbase=110000  Vref=1  Vangle=0  VLF=1  angleLF=0
      settings: AttributesFormatString=|
      | %<ID>
      | %<Vbase>V
      | %<VLF>pu
      | %<angleLF>deg.
      | %<Name>
  bus173 : powerlib/Measurements/Load Flow Bus  LConnTagsString=a  ID=bus173  Vbase=110000  Vref=1  Vangle=0  VLF=1  angleLF=0
      settings: AttributesFormatString=|
      | %<ID>
      | %<Vbase>V
      | %<VLF>pu
      | %<angleLF>deg.
      | %<Name>
  bus174 : powerlib/Measurements/Load Flow Bus  LConnTagsString=a  ID=bus174  Vbase=110000  Vref=1  Vangle=0  VLF=1  angleLF=0
      settings: AttributesFormatString=|
      | %<ID>
      | %<Vbase>V
      | %<VLF>pu
      | %<angleLF>deg.
      | %<Name>
  bus175 : powerlib/Measurements/Load Flow Bus  LConnTagsString=a  ID=bus175  Vbase=110000  Vref=1  Vangle=0  VLF=1  angleLF=0
      settings: AttributesFormatString=|
      | %<ID>
      | %<Vbase>V
      | %<VLF>pu
      | %<angleLF>deg.
      | %<Name>
  bus176 : powerlib/Measurements/Load Flow Bus  LConnTagsString=a  ID=bus176  Vbase=110000  Vref=1  Vangle=0  VLF=1  angleLF=0
      settings: AttributesFormatString=|
      | %<ID>
      | %<Vbase>V
      | %<VLF>pu
      | %<angleLF>deg.
      | %<Name>
  bus177 : powerlib/Measurements/Load Flow Bus  LConnTagsString=a  ID=bus177  Vbase=110000  Vref=1  Vangle=0  VLF=1  angleLF=0
      settings: AttributesFormatString=|
      | %<ID>
      | %<Vbase>V
      | %<VLF>pu
      | %<angleLF>deg.
      | %<Name>
  bus178 : powerlib/Measurements/Load Flow Bus  LConnTagsString=a  ID=bus178  Vbase=110000  Vref=1  Vangle=0  VLF=1  angleLF=0
      settings: AttributesFormatString=|
      | %<ID>
      | %<Vbase>V
      | %<VLF>pu
      | %<angleLF>deg.
      | %<Name>
  bus179 : powerlib/Measurements/Load Flow Bus  LConnTagsString=a  ID=bus179  Vbase=110000  Vref=1  Vangle=0  VLF=1  angleLF=0
      settings: AttributesFormatString=|
      | %<ID>
      | %<Vbase>V
      | %<VLF>pu
      | %<angleLF>deg.
      | %<Name>
  bus18 : powerlib/Measurements/Load Flow Bus  LConnTagsString=a  ID=bus18  Vbase=110000  Vref=1  Vangle=0  VLF=1  angleLF=0
      settings: AttributesFormatString=|
      | %<ID>
      | %<Vbase>V
      | %<VLF>pu
      | %<angleLF>deg.
      | %<Name>
  bus180 : powerlib/Measurements/Load Flow Bus  LConnTagsString=a  ID=bus180  Vbase=110000  Vref=1  Vangle=0  VLF=1  angleLF=0
      settings: AttributesFormatString=|
      | %<ID>
      | %<Vbase>V
      | %<VLF>pu
      | %<angleLF>deg.
      | %<Name>
  bus181 : powerlib/Measurements/Load Flow Bus  LConnTagsString=a  ID=bus181  Vbase=110000  Vref=1  Vangle=0  VLF=1  angleLF=0
      settings: AttributesFormatString=|
      | %<ID>
      | %<Vbase>V
      | %<VLF>pu
      | %<angleLF>deg.
      | %<Name>
  bus182 : powerlib/Measurements/Load Flow Bus  LConnTagsString=a  ID=bus182  Vbase=110000  Vref=1  Vangle=0  VLF=1  angleLF=0
      settings: AttributesFormatString=|
      | %<ID>
      | %<Vbase>V
      | %<VLF>pu
      | %<angleLF>deg.
      | %<Name>
  bus183 : powerlib/Measurements/Load Flow Bus  LConnTagsString=a  ID=bus183  Vbase=110000  Vref=1  Vangle=0  VLF=1  angleLF=0
      settings: AttributesFormatString=|
      | %<ID>
      | %<Vbase>V
      | %<VLF>pu
      | %<angleLF>deg.
      | %<Name>
  bus184 : powerlib/Measurements/Load Flow Bus  LConnTagsString=a  ID=bus184  Vbase=110000  Vref=1  Vangle=0  VLF=1  angleLF=0
      settings: AttributesFormatString=|
      | %<ID>
      | %<Vbase>V
      | %<VLF>pu
      | %<angleLF>deg.
      | %<Name>
  bus185 : powerlib/Measurements/Load Flow Bus  LConnTagsString=a  ID=bus185  Vbase=110000  Vref=1  Vangle=0  VLF=1  angleLF=0
      settings: AttributesFormatString=|
      | %<ID>
      | %<Vbase>V
      | %<VLF>pu
      | %<angleLF>deg.
      | %<Name>
  bus186 : powerlib/Measurements/Load Flow Bus  LConnTagsString=a  ID=bus186  Vbase=110000  Vref=1  Vangle=0  VLF=1  angleLF=0
      settings: AttributesFormatString=|
      | %<ID>
      | %<Vbase>V
      | %<VLF>pu
      | %<angleLF>deg.
      | %<Name>
  bus187 : powerlib/Measurements/Load Flow Bus  LConnTagsString=a  ID=bus187  Vbase=110000  Vref=1  Vangle=0  VLF=1  angleLF=0
      settings: AttributesFormatString=|
      | %<ID>
      | %<Vbase>V
      | %<VLF>pu
      | %<angleLF>deg.
      | %<Name>
  bus188 : powerlib/Measurements/Load Flow Bus  LConnTagsString=a  ID=bus188  Vbase=110000  Vref=1  Vangle=0  VLF=1  angleLF=0
      settings: AttributesFormatString=|
      | %<ID>
      | %<Vbase>V
      | %<VLF>pu
      | %<angleLF>deg.
      | %<Name>
  bus189 : powerlib/Measurements/Load Flow Bus  LConnTagsString=a  ID=bus189  Vbase=110000  Vref=1  Vangle=0  VLF=1  angleLF=0
      settings: AttributesFormatString=|
      | %<ID>
      | %<Vbase>V
      | %<VLF>pu
      | %<angleLF>deg.
      | %<Name>
  bus19 : powerlib/Measurements/Load Flow Bus  LConnTagsString=a  ID=bus19  Vbase=110000  Vref=1  Vangle=0  VLF=1  angleLF=0
      settings: AttributesFormatString=|
      | %<ID>
      | %<Vbase>V
      | %<VLF>pu
      | %<angleLF>deg.
      | %<Name>
  bus190 : powerlib/Measurements/Load Flow Bus  LConnTagsString=a  ID=bus190  Vbase=110000  Vref=1  Vangle=0  VLF=1  angleLF=0
      settings: AttributesFormatString=|
      | %<ID>
      | %<Vbase>V
      | %<VLF>pu
      | %<angleLF>deg.
      | %<Name>
  bus191 : powerlib/Measurements/Load Flow Bus  LConnTagsString=a  ID=bus191  Vbase=110000  Vref=1  Vangle=0  VLF=1  angleLF=0
      settings: AttributesFormatString=|
      | %<ID>
      | %<Vbase>V
      | %<VLF>pu
      | %<angleLF>deg.
      | %<Name>
  bus192 : powerlib/Measurements/Load Flow Bus  LConnTagsString=a  ID=bus192  Vbase=110000  Vref=1  Vangle=0  VLF=1  angleLF=0
      settings: AttributesFormatString=|
      | %<ID>
      | %<Vbase>V
      | %<VLF>pu
      | %<angleLF>deg.
      | %<Name>
  bus193 : powerlib/Measurements/Load Flow Bus  LConnTagsString=a  ID=bus193  Vbase=110000  Vref=1  Vangle=0  VLF=1  angleLF=0
      settings: AttributesFormatString=|
      | %<ID>
      | %<Vbase>V
      | %<VLF>pu
      | %<angleLF>deg.
      | %<Name>
  bus194 : powerlib/Measurements/Load Flow Bus  LConnTagsString=a  ID=bus194  Vbase=110000  Vref=1  Vangle=0  VLF=1  angleLF=0
      settings: AttributesFormatString=|
      | %<ID>
      | %<Vbase>V
      | %<VLF>pu
      | %<angleLF>deg.
      | %<Name>
  bus195 : powerlib/Measurements/Load Flow Bus  LConnTagsString=a  ID=bus195  Vbase=110000  Vref=1  Vangle=0  VLF=1  angleLF=0
      settings: AttributesFormatString=|
      | %<ID>
      | %<Vbase>V
      | %<VLF>pu
      | %<angleLF>deg.
      | %<Name>
  bus196 : powerlib/Measurements/Load Flow Bus  LConnTagsString=a  ID=bus196  Vbase=110000  Vref=1  Vangle=0  VLF=1  angleLF=0
      settings: AttributesFormatString=|
      | %<ID>
      | %<Vbase>V
      | %<VLF>pu
      | %<angleLF>deg.
      | %<Name>
  bus197 : powerlib/Measurements/Load Flow Bus  LConnTagsString=a  ID=bus197  Vbase=110000  Vref=1  Vangle=0  VLF=1  angleLF=0
      settings: AttributesFormatString=|
      | %<ID>
      | %<Vbase>V
      | %<VLF>pu
      | %<angleLF>deg.
      | %<Name>
  bus198 : powerlib/Measurements/Load Flow Bus  LConnTagsString=a  ID=bus198  Vbase=110000  Vref=1  Vangle=0  VLF=1  angleLF=0
      settings: AttributesFormatString=|
      | %<ID>
      | %<Vbase>V
      | %<VLF>pu
      | %<angleLF>deg.
      | %<Name>
  bus199 : powerlib/Measurements/Load Flow Bus  LConnTagsString=a  ID=bus199  Vbase=110000  Vref=1  Vangle=0  VLF=1  angleLF=0
      settings: AttributesFormatString=|
      | %<ID>
      | %<Vbase>V
      | %<VLF>pu
      | %<angleLF>deg.
      | %<Name>
  bus2 : powerlib/Measurements/Load Flow Bus  LConnTagsString=a  ID=bus2  Vbase=110000  Vref=1  Vangle=0  VLF=1  angleLF=0
      settings: AttributesFormatString=|
      | %<ID>
      | %<Vbase>V
      | %<VLF>pu
      | %<angleLF>deg.
      | %<Name>
  bus20 : powerlib/Measurements/Load Flow Bus  LConnTagsString=a  ID=bus20  Vbase=110000  Vref=1  Vangle=0  VLF=1  angleLF=0
      settings: AttributesFormatString=|
      | %<ID>
      | %<Vbase>V
      | %<VLF>pu
      | %<angleLF>deg.
      | %<Name>
  bus200 : powerlib/Measurements/Load Flow Bus  LConnTagsString=a  ID=bus200  Vbase=110000  Vref=1  Vangle=0  VLF=1  angleLF=0
      settings: AttributesFormatString=|
      | %<ID>
      | %<Vbase>V
      | %<VLF>pu
      | %<angleLF>deg.
      | %<Name>
  bus201 : powerlib/Measurements/Load Flow Bus  LConnTagsString=a  ID=bus201  Vbase=110000  Vref=1  Vangle=0  VLF=1  angleLF=0
      settings: AttributesFormatString=|
      | %<ID>
      | %<Vbase>V
      | %<VLF>pu
      | %<angleLF>deg.
      | %<Name>
  bus202 : powerlib/Measurements/Load Flow Bus  LConnTagsString=a  ID=bus202  Vbase=110000  Vref=1  Vangle=0  VLF=1  angleLF=0
      settings: AttributesFormatString=|
      | %<ID>
      | %<Vbase>V
      | %<VLF>pu
      | %<angleLF>deg.
      | %<Name>
  bus203 : powerlib/Measurements/Load Flow Bus  LConnTagsString=a  ID=bus203  Vbase=110000  Vref=1  Vangle=0  VLF=1  angleLF=0
      settings: AttributesFormatString=|
      | %<ID>
      | %<Vbase>V
      | %<VLF>pu
      | %<angleLF>deg.
      | %<Name>
  bus204 : powerlib/Measurements/Load Flow Bus  LConnTagsString=a  ID=bus204  Vbase=110000  Vref=1  Vangle=0  VLF=1  angleLF=0
      settings: AttributesFormatString=|
      | %<ID>
      | %<Vbase>V
      | %<VLF>pu
      | %<angleLF>deg.
      | %<Name>
  bus205 : powerlib/Measurements/Load Flow Bus  LConnTagsString=a  ID=bus205  Vbase=110000  Vref=1  Vangle=0  VLF=1  angleLF=0
      settings: AttributesFormatString=|
      | %<ID>
      | %<Vbase>V
      | %<VLF>pu
      | %<angleLF>deg.
      | %<Name>
  bus206 : powerlib/Measurements/Load Flow Bus  LConnTagsString=a  ID=bus206  Vbase=110000  Vref=1  Vangle=0  VLF=1  angleLF=0
      settings: AttributesFormatString=|
      | %<ID>
      | %<Vbase>V
      | %<VLF>pu
      | %<angleLF>deg.
      | %<Name>
  bus207 : powerlib/Measurements/Load Flow Bus  LConnTagsString=a  ID=bus207  Vbase=110000  Vref=1  Vangle=0  VLF=1  angleLF=0
      settings: AttributesFormatString=|
      | %<ID>
      | %<Vbase>V
      | %<VLF>pu
      | %<angleLF>deg.
      | %<Name>
  bus208 : powerlib/Measurements/Load Flow Bus  LConnTagsString=a  ID=bus208  Vbase=110000  Vref=1  Vangle=0  VLF=1  angleLF=0
      settings: AttributesFormatString=|
      | %<ID>
      | %<Vbase>V
      | %<VLF>pu
      | %<angleLF>deg.
      | %<Name>
  bus209 : powerlib/Measurements/Load Flow Bus  LConnTagsString=a  ID=bus209  Vbase=110000  Vref=1  Vangle=0  VLF=1  angleLF=0
      settings: AttributesFormatString=|
      | %<ID>
      | %<Vbase>V
      | %<VLF>pu
      | %<angleLF>deg.
      | %<Name>
  bus21 : powerlib/Measurements/Load Flow Bus  LConnTagsString=a  ID=bus21  Vbase=110000  Vref=1  Vangle=0  VLF=1  angleLF=0
      settings: AttributesFormatString=|
      | %<ID>
      | %<Vbase>V
      | %<VLF>pu
      | %<angleLF>deg.
      | %<Name>
  bus210 : powerlib/Measurements/Load Flow Bus  LConnTagsString=a  ID=bus210  Vbase=110000  Vref=1  Vangle=0  VLF=1  angleLF=0
      settings: AttributesFormatString=|
      | %<ID>
      | %<Vbase>V
      | %<VLF>pu
      | %<angleLF>deg.
      | %<Name>
  bus211 : powerlib/Measurements/Load Flow Bus  LConnTagsString=a  ID=bus211  Vbase=110000  Vref=1  Vangle=0  VLF=1  angleLF=0
      settings: AttributesFormatString=|
      | %<ID>
      | %<Vbase>V
      | %<VLF>pu
      | %<angleLF>deg.
      | %<Name>
  bus212 : powerlib/Measurements/Load Flow Bus  LConnTagsString=a  ID=bus212  Vbase=110000  Vref=1  Vangle=0  VLF=1  angleLF=0
      settings: AttributesFormatString=|
      | %<ID>
      | %<Vbase>V
      | %<VLF>pu
      | %<angleLF>deg.
      | %<Name>
  bus213 : powerlib/Measurements/Load Flow Bus  LConnTagsString=a  ID=bus213  Vbase=110000  Vref=1  Vangle=0  VLF=1  angleLF=0
      settings: AttributesFormatString=|
      | %<ID>
      | %<Vbase>V
      | %<VLF>pu
      | %<angleLF>deg.
      | %<Name>
  bus214 : powerlib/Measurements/Load Flow Bus  LConnTagsString=a  ID=bus214  Vbase=110000  Vref=1  Vangle=0  VLF=1  angleLF=0
      settings: AttributesFormatString=|
      | %<ID>
      | %<Vbase>V
      | %<VLF>pu
      | %<angleLF>deg.
      | %<Name>
  bus215 : powerlib/Measurements/Load Flow Bus  LConnTagsString=a  ID=bus215  Vbase=110000  Vref=1  Vangle=0  VLF=1  angleLF=0
      settings: AttributesFormatString=|
      | %<ID>
      | %<Vbase>V
      | %<VLF>pu
      | %<angleLF>deg.
      | %<Name>
  bus216 : powerlib/Measurements/Load Flow Bus  LConnTagsString=a  ID=bus216  Vbase=110000  Vref=1  Vangle=0  VLF=1  angleLF=0
      settings: AttributesFormatString=|
      | %<ID>
      | %<Vbase>V
      | %<VLF>pu
      | %<angleLF>deg.
      | %<Name>
  bus217 : powerlib/Measurements/Load Flow Bus  LConnTagsString=a  ID=bus217  Vbase=110000  Vref=1  Vangle=0  VLF=1  angleLF=0
      settings: AttributesFormatString=|
      | %<ID>
      | %<Vbase>V
      | %<VLF>pu
      | %<angleLF>deg.
      | %<Name>
  bus218 : powerlib/Measurements/Load Flow Bus  LConnTagsString=a  ID=bus218  Vbase=110000  Vref=1  Vangle=0  VLF=1  angleLF=0
      settings: AttributesFormatString=|
      | %<ID>
      | %<Vbase>V
      | %<VLF>pu
      | %<angleLF>deg.
      | %<Name>
  bus219 : powerlib/Measurements/Load Flow Bus  LConnTagsString=a  ID=bus219  Vbase=110000  Vref=1  Vangle=0  VLF=1  angleLF=0
      settings: AttributesFormatString=|
      | %<ID>
      | %<Vbase>V
      | %<VLF>pu
      | %<angleLF>deg.
      | %<Name>
  bus22 : powerlib/Measurements/Load Flow Bus  LConnTagsString=a  ID=bus22  Vbase=110000  Vref=1  Vangle=0  VLF=1  angleLF=0
      settings: AttributesFormatString=|
      | %<ID>
      | %<Vbase>V
      | %<VLF>pu
      | %<angleLF>deg.
      | %<Name>
  bus220 : powerlib/Measurements/Load Flow Bus  LConnTagsString=a  ID=bus220  Vbase=110000  Vref=1  Vangle=0  VLF=1  angleLF=0
      settings: AttributesFormatString=|
      | %<ID>
      | %<Vbase>V
      | %<VLF>pu
      | %<angleLF>deg.
      | %<Name>
  bus221 : powerlib/Measurements/Load Flow Bus  LConnTagsString=a  ID=bus221  Vbase=110000  Vref=1  Vangle=0  VLF=1  angleLF=0
      settings: AttributesFormatString=|
      | %<ID>
      | %<Vbase>V
      | %<VLF>pu
      | %<angleLF>deg.
      | %<Name>
  bus222 : powerlib/Measurements/Load Flow Bus  LConnTagsString=a  ID=bus222  Vbase=110000  Vref=1  Vangle=0  VLF=1  angleLF=0
      settings: AttributesFormatString=|
      | %<ID>
      | %<Vbase>V
      | %<VLF>pu
      | %<angleLF>deg.
      | %<Name>
  bus223 : powerlib/Measurements/Load Flow Bus  LConnTagsString=a  ID=bus223  Vbase=110000  Vref=1  Vangle=0  VLF=1  angleLF=0
      settings: AttributesFormatString=|
      | %<ID>
      | %<Vbase>V
      | %<VLF>pu
      | %<angleLF>deg.
      | %<Name>
  bus224 : powerlib/Measurements/Load Flow Bus  LConnTagsString=a  ID=bus224  Vbase=110000  Vref=1  Vangle=0  VLF=1  angleLF=0
      settings: AttributesFormatString=|
      | %<ID>
      | %<Vbase>V
      | %<VLF>pu
      | %<angleLF>deg.
      | %<Name>
  bus225 : powerlib/Measurements/Load Flow Bus  LConnTagsString=a  ID=bus225  Vbase=110000  Vref=1  Vangle=0  VLF=1  angleLF=0
      settings: AttributesFormatString=|
      | %<ID>
      | %<Vbase>V
      | %<VLF>pu
      | %<angleLF>deg.
      | %<Name>
  bus226 : powerlib/Measurements/Load Flow Bus  LConnTagsString=a  ID=bus226  Vbase=110000  Vref=1  Vangle=0  VLF=1  angleLF=0
      settings: AttributesFormatString=|
      | %<ID>
      | %<Vbase>V
      | %<VLF>pu
      | %<angleLF>deg.
      | %<Name>
  bus227 : powerlib/Measurements/Load Flow Bus  LConnTagsString=a  ID=bus227  Vbase=110000  Vref=1  Vangle=0  VLF=1  angleLF=0
      settings: AttributesFormatString=|
      | %<ID>
      | %<Vbase>V
      | %<VLF>pu
      | %<angleLF>deg.
      | %<Name>
  bus228 : powerlib/Measurements/Load Flow Bus  LConnTagsString=a  ID=bus228  Vbase=110000  Vref=1  Vangle=0  VLF=1  angleLF=0
      settings: AttributesFormatString=|
      | %<ID>
      | %<Vbase>V
      | %<VLF>pu
      | %<angleLF>deg.
      | %<Name>
  bus229 : powerlib/Measurements/Load Flow Bus  LConnTagsString=a  ID=bus229  Vbase=110000  Vref=1  Vangle=0  VLF=1  angleLF=0
      settings: AttributesFormatString=|
      | %<ID>
      | %<Vbase>V
      | %<VLF>pu
      | %<angleLF>deg.
      | %<Name>
  bus23 : powerlib/Measurements/Load Flow Bus  LConnTagsString=a  ID=bus23  Vbase=110000  Vref=1  Vangle=0  VLF=1  angleLF=0
      settings: AttributesFormatString=|
      | %<ID>
      | %<Vbase>V
      | %<VLF>pu
      | %<angleLF>deg.
      | %<Name>
  bus230 : powerlib/Measurements/Load Flow Bus  LConnTagsString=a  ID=bus230  Vbase=110000  Vref=1  Vangle=0  VLF=1  angleLF=0
      settings: AttributesFormatString=|
      | %<ID>
      | %<Vbase>V
      | %<VLF>pu
      | %<angleLF>deg.
      | %<Name>
  bus231 : powerlib/Measurements/Load Flow Bus  LConnTagsString=a  ID=bus231  Vbase=110000  Vref=1  Vangle=0  VLF=1  angleLF=0
      settings: AttributesFormatString=|
      | %<ID>
      | %<Vbase>V
      | %<VLF>pu
      | %<angleLF>deg.
      | %<Name>
  bus232 : powerlib/Measurements/Load Flow Bus  LConnTagsString=a  ID=bus232  Vbase=110000  Vref=1  Vangle=0  VLF=1  angleLF=0
      settings: AttributesFormatString=|
      | %<ID>
      | %<Vbase>V
      | %<VLF>pu
      | %<angleLF>deg.
      | %<Name>
  bus233 : powerlib/Measurements/Load Flow Bus  LConnTagsString=a  ID=bus233  Vbase=110000  Vref=1  Vangle=0  VLF=1  angleLF=0
      settings: AttributesFormatString=|
      | %<ID>
      | %<Vbase>V
      | %<VLF>pu
      | %<angleLF>deg.
      | %<Name>
  bus234 : powerlib/Measurements/Load Flow Bus  LConnTagsString=a  ID=bus234  Vbase=110000  Vref=1  Vangle=0  VLF=1  angleLF=0
      settings: AttributesFormatString=|
      | %<ID>
      | %<Vbase>V
      | %<VLF>pu
      | %<angleLF>deg.
      | %<Name>
  bus235 : powerlib/Measurements/Load Flow Bus  LConnTagsString=a  ID=bus235  Vbase=110000  Vref=1  Vangle=0  VLF=1  angleLF=0
      settings: AttributesFormatString=|
      | %<ID>
      | %<Vbase>V
      | %<VLF>pu
      | %<angleLF>deg.
      | %<Name>
  bus236 : powerlib/Measurements/Load Flow Bus  LConnTagsString=a  ID=bus236  Vbase=110000  Vref=1  Vangle=0  VLF=1  angleLF=0
      settings: AttributesFormatString=|
      | %<ID>
      | %<Vbase>V
      | %<VLF>pu
      | %<angleLF>deg.
      | %<Name>
  bus237 : powerlib/Measurements/Load Flow Bus  LConnTagsString=a  ID=bus237  Vbase=110000  Vref=1  Vangle=0  VLF=1  angleLF=0
      settings: AttributesFormatString=|
      | %<ID>
      | %<Vbase>V
      | %<VLF>pu
      | %<angleLF>deg.
      | %<Name>
  bus238 : powerlib/Measurements/Load Flow Bus  LConnTagsString=a  ID=bus238  Vbase=110000  Vref=1  Vangle=0  VLF=1  angleLF=0
      settings: AttributesFormatString=|
      | %<ID>
      | %<Vbase>V
      | %<VLF>pu
      | %<angleLF>deg.
      | %<Name>
  bus239 : powerlib/Measurements/Load Flow Bus  LConnTagsString=a  ID=bus239  Vbase=110000  Vref=1  Vangle=0  VLF=1  angleLF=0
      settings: AttributesFormatString=|
      | %<ID>
      | %<Vbase>V
      | %<VLF>pu
      | %<angleLF>deg.
      | %<Name>
  bus24 : powerlib/Measurements/Load Flow Bus  LConnTagsString=a  ID=bus24  Vbase=110000  Vref=1  Vangle=0  VLF=1  angleLF=0
      settings: AttributesFormatString=|
      | %<ID>
      | %<Vbase>V
      | %<VLF>pu
      | %<angleLF>deg.
      | %<Name>
  bus240 : powerlib/Measurements/Load Flow Bus  LConnTagsString=a  ID=bus240  Vbase=110000  Vref=1  Vangle=0  VLF=1  angleLF=0
      settings: AttributesFormatString=|
      | %<ID>
      | %<Vbase>V
      | %<VLF>pu
      | %<angleLF>deg.
      | %<Name>
  bus241 : powerlib/Measurements/Load Flow Bus  LConnTagsString=a  ID=bus241  Vbase=110000  Vref=1  Vangle=0  VLF=1  angleLF=0
      settings: AttributesFormatString=|
      | %<ID>
      | %<Vbase>V
      | %<VLF>pu
      | %<angleLF>deg.
      | %<Name>
  bus242 : powerlib/Measurements/Load Flow Bus  LConnTagsString=a  ID=bus242  Vbase=110000  Vref=1  Vangle=0  VLF=1  angleLF=0
      settings: AttributesFormatString=|
      | %<ID>
      | %<Vbase>V
      | %<VLF>pu
      | %<angleLF>deg.
      | %<Name>
  bus243 : powerlib/Measurements/Load Flow Bus  LConnTagsString=a  ID=bus243  Vbase=110000  Vref=1  Vangle=0  VLF=1  angleLF=0
      settings: AttributesFormatString=|
      | %<ID>
      | %<Vbase>V
      | %<VLF>pu
      | %<angleLF>deg.
      | %<Name>
  bus244 : powerlib/Measurements/Load Flow Bus  LConnTagsString=a  ID=bus244  Vbase=110000  Vref=1  Vangle=0  VLF=1  angleLF=0
      settings: AttributesFormatString=|
      | %<ID>
      | %<Vbase>V
      | %<VLF>pu
      | %<angleLF>deg.
      | %<Name>
  bus245 : powerlib/Measurements/Load Flow Bus  LConnTagsString=a  ID=bus245  Vbase=110000  Vref=1  Vangle=0  VLF=1  angleLF=0
      settings: AttributesFormatString=|
      | %<ID>
      | %<Vbase>V
      | %<VLF>pu
      | %<angleLF>deg.
      | %<Name>
  bus246 : powerlib/Measurements/Load Flow Bus  LConnTagsString=a  ID=bus246  Vbase=110000  Vref=1  Vangle=0  VLF=1  angleLF=0
      settings: AttributesFormatString=|
      | %<ID>
      | %<Vbase>V
      | %<VLF>pu
      | %<angleLF>deg.
      | %<Name>
  bus247 : powerlib/Measurements/Load Flow Bus  LConnTagsString=a  ID=bus247  Vbase=220000  Vref=1  Vangle=0  VLF=1  angleLF=0
      settings: AttributesFormatString=|
      | %<ID>
      | %<Vbase>V
      | %<VLF>pu
      | %<angleLF>deg.
      | %<Name>
  bus248 : powerlib/Measurements/Load Flow Bus  LConnTagsString=a  ID=bus248  Vbase=220000  Vref=1  Vangle=0  VLF=1  angleLF=0
      settings: AttributesFormatString=|
      | %<ID>
      | %<Vbase>V
      | %<VLF>pu
      | %<angleLF>deg.
      | %<Name>
  bus249 : powerlib/Measurements/Load Flow Bus  LConnTagsString=a  ID=bus249  Vbase=220000  Vref=1  Vangle=0  VLF=1  angleLF=0
      settings: AttributesFormatString=|
      | %<ID>
      | %<Vbase>V
      | %<VLF>pu
      | %<angleLF>deg.
      | %<Name>
  bus25 : powerlib/Measurements/Load Flow Bus  LConnTagsString=a  ID=bus25  Vbase=110000  Vref=1  Vangle=0  VLF=1  angleLF=0
      settings: AttributesFormatString=|
      | %<ID>
      | %<Vbase>V
      | %<VLF>pu
      | %<angleLF>deg.
      | %<Name>
  bus250 : powerlib/Measurements/Load Flow Bus  LConnTagsString=a  ID=bus250  Vbase=220000  Vref=1  Vangle=0  VLF=1  angleLF=0
      settings: AttributesFormatString=|
      | %<ID>
      | %<Vbase>V
      | %<VLF>pu
      | %<angleLF>deg.
      | %<Name>
  bus251 : powerlib/Measurements/Load Flow Bus  LConnTagsString=a  ID=bus251  Vbase=220000  Vref=1  Vangle=0  VLF=1  angleLF=0
      settings: AttributesFormatString=|
      | %<ID>
      | %<Vbase>V
      | %<VLF>pu
      | %<angleLF>deg.
      | %<Name>
  bus252 : powerlib/Measurements/Load Flow Bus  LConnTagsString=a  ID=bus252  Vbase=220000  Vref=1  Vangle=0  VLF=1  angleLF=0
      settings: AttributesFormatString=|
      | %<ID>
      | %<Vbase>V
      | %<VLF>pu
      | %<angleLF>deg.
      | %<Name>
  bus253 : powerlib/Measurements/Load Flow Bus  LConnTagsString=a  ID=bus253  Vbase=220000  Vref=1  Vangle=0  VLF=1  angleLF=0
      settings: AttributesFormatString=|
      | %<ID>
      | %<Vbase>V
      | %<VLF>pu
      | %<angleLF>deg.
      | %<Name>
  bus254 : powerlib/Measurements/Load Flow Bus  LConnTagsString=a  ID=bus254  Vbase=220000  Vref=1  Vangle=0  VLF=1  angleLF=0
      settings: AttributesFormatString=|
      | %<ID>
      | %<Vbase>V
      | %<VLF>pu
      | %<angleLF>deg.
      | %<Name>
  bus255 : powerlib/Measurements/Load Flow Bus  LConnTagsString=a  ID=bus255  Vbase=220000  Vref=1  Vangle=0  VLF=1  angleLF=0
      settings: AttributesFormatString=|
      | %<ID>
      | %<Vbase>V
      | %<VLF>pu
      | %<angleLF>deg.
      | %<Name>
  bus256 : powerlib/Measurements/Load Flow Bus  LConnTagsString=a  ID=bus256  Vbase=220000  Vref=1  Vangle=0  VLF=1  angleLF=0
      settings: AttributesFormatString=|
      | %<ID>
      | %<Vbase>V
      | %<VLF>pu
      | %<angleLF>deg.
      | %<Name>
  bus257 : powerlib/Measurements/Load Flow Bus  LConnTagsString=a  ID=bus257  Vbase=220000  Vref=1  Vangle=0  VLF=1  angleLF=0
      settings: AttributesFormatString=|
      | %<ID>
      | %<Vbase>V
      | %<VLF>pu
      | %<angleLF>deg.
      | %<Name>
  bus258 : powerlib/Measurements/Load Flow Bus  LConnTagsString=a  ID=bus258  Vbase=220000  Vref=1  Vangle=0  VLF=1  angleLF=0
      settings: AttributesFormatString=|
      | %<ID>
      | %<Vbase>V
      | %<VLF>pu
      | %<angleLF>deg.
      | %<Name>
  bus259 : powerlib/Measurements/Load Flow Bus  LConnTagsString=a  ID=bus259  Vbase=220000  Vref=1  Vangle=0  VLF=1  angleLF=0
      settings: AttributesFormatString=|
      | %<ID>
      | %<Vbase>V
      | %<VLF>pu
      | %<angleLF>deg.
      | %<Name>
  bus26 : powerlib/Measurements/Load Flow Bus  LConnTagsString=a  ID=bus26  Vbase=110000  Vref=1  Vangle=0  VLF=1  angleLF=0
      settings: AttributesFormatString=|
      | %<ID>
      | %<Vbase>V
      | %<VLF>pu
      | %<angleLF>deg.
      | %<Name>
  bus260 : powerlib/Measurements/Load Flow Bus  LConnTagsString=a  ID=bus260  Vbase=220000  Vref=1  Vangle=0  VLF=1  angleLF=0
      settings: AttributesFormatString=|
      | %<ID>
      | %<Vbase>V
      | %<VLF>pu
      | %<angleLF>deg.
      | %<Name>
  bus261 : powerlib/Measurements/Load Flow Bus  LConnTagsString=a  ID=bus261  Vbase=220000  Vref=1  Vangle=0  VLF=1  angleLF=0
      settings: AttributesFormatString=|
      | %<ID>
      | %<Vbase>V
      | %<VLF>pu
      | %<angleLF>deg.
      | %<Name>
  bus262 : powerlib/Measurements/Load Flow Bus  LConnTagsString=a  ID=bus262  Vbase=220000  Vref=1  Vangle=0  VLF=1  angleLF=0
      settings: AttributesFormatString=|
      | %<ID>
      | %<Vbase>V
      | %<VLF>pu
      | %<angleLF>deg.
      | %<Name>
  bus263 : powerlib/Measurements/Load Flow Bus  LConnTagsString=a  ID=bus263  Vbase=220000  Vref=1  Vangle=0  VLF=1  angleLF=0
      settings: AttributesFormatString=|
      | %<ID>
      | %<Vbase>V
      | %<VLF>pu
      | %<angleLF>deg.
      | %<Name>
  bus264 : powerlib/Measurements/Load Flow Bus  LConnTagsString=a  ID=bus264  Vbase=220000  Vref=1  Vangle=0  VLF=1  angleLF=0
      settings: AttributesFormatString=|
      | %<ID>
      | %<Vbase>V
      | %<VLF>pu
      | %<angleLF>deg.
      | %<Name>
  bus265 : powerlib/Measurements/Load Flow Bus  LConnTagsString=a  ID=bus265  Vbase=220000  Vref=1  Vangle=0  VLF=1  angleLF=0
      settings: AttributesFormatString=|
      | %<ID>
      | %<Vbase>V
      | %<VLF>pu
      | %<angleLF>deg.
      | %<Name>
  bus266 : powerlib/Measurements/Load Flow Bus  LConnTagsString=a  ID=bus266  Vbase=220000  Vref=1  Vangle=0  VLF=1  angleLF=0
      settings: AttributesFormatString=|
      | %<ID>
      | %<Vbase>V
      | %<VLF>pu
      | %<angleLF>deg.
      | %<Name>
  bus267 : powerlib/Measurements/Load Flow Bus  LConnTagsString=a  ID=bus267  Vbase=220000  Vref=1  Vangle=0  VLF=1  angleLF=0
      settings: AttributesFormatString=|
      | %<ID>
      | %<Vbase>V
      | %<VLF>pu
      | %<angleLF>deg.
      | %<Name>
  bus268 : powerlib/Measurements/Load Flow Bus  LConnTagsString=a  ID=bus268  Vbase=220000  Vref=1  Vangle=0  VLF=1  angleLF=0
      settings: AttributesFormatString=|
      | %<ID>
      | %<Vbase>V
      | %<VLF>pu
      | %<angleLF>deg.
      | %<Name>
  bus269 : powerlib/Measurements/Load Flow Bus  LConnTagsString=a  ID=bus269  Vbase=220000  Vref=1  Vangle=0  VLF=1  angleLF=0
      settings: AttributesFormatString=|
      | %<ID>
      | %<Vbase>V
      | %<VLF>pu
      | %<angleLF>deg.
      | %<Name>
  bus27 : powerlib/Measurements/Load Flow Bus  LConnTagsString=a  ID=bus27  Vbase=110000  Vref=1  Vangle=0  VLF=1  angleLF=0
      settings: AttributesFormatString=|
      | %<ID>
      | %<Vbase>V
      | %<VLF>pu
      | %<angleLF>deg.
      | %<Name>
  bus270 : powerlib/Measurements/Load Flow Bus  LConnTagsString=a  ID=bus270  Vbase=220000  Vref=1  Vangle=0  VLF=1  angleLF=0
      settings: AttributesFormatString=|
      | %<ID>
      | %<Vbase>V
      | %<VLF>pu
      | %<angleLF>deg.
      | %<Name>
  bus271 : powerlib/Measurements/Load Flow Bus  LConnTagsString=a  ID=bus271  Vbase=220000  Vref=1  Vangle=0  VLF=1  angleLF=0
      settings: AttributesFormatString=|
      | %<ID>
      | %<Vbase>V
      | %<VLF>pu
      | %<angleLF>deg.
      | %<Name>
  bus272 : powerlib/Measurements/Load Flow Bus  LConnTagsString=a  ID=bus272  Vbase=220000  Vref=1  Vangle=0  VLF=1  angleLF=0
      settings: AttributesFormatString=|
      | %<ID>
      | %<Vbase>V
      | %<VLF>pu
      | %<angleLF>deg.
      | %<Name>
  bus273 : powerlib/Measurements/Load Flow Bus  LConnTagsString=a  ID=bus273  Vbase=220000  Vref=1  Vangle=0  VLF=1  angleLF=0
      settings: AttributesFormatString=|
      | %<ID>
      | %<Vbase>V
      | %<VLF>pu
      | %<angleLF>deg.
      | %<Name>
  bus274 : powerlib/Measurements/Load Flow Bus  LConnTagsString=a  ID=bus274  Vbase=220000  Vref=1  Vangle=0  VLF=1  angleLF=0
      settings: AttributesFormatString=|
      | %<ID>
      | %<Vbase>V
      | %<VLF>pu
      | %<angleLF>deg.
      | %<Name>
  bus275 : powerlib/Measurements/Load Flow Bus  LConnTagsString=a  ID=bus275  Vbase=220000  Vref=1  Vangle=0  VLF=1  angleLF=0
      settings: AttributesFormatString=|
      | %<ID>
      | %<Vbase>V
      | %<VLF>pu
      | %<angleLF>deg.
      | %<Name>
  bus276 : powerlib/Measurements/Load Flow Bus  LConnTagsString=a  ID=bus276  Vbase=220000  Vref=1  Vangle=0  VLF=1  angleLF=0
      settings: AttributesFormatString=|
      | %<ID>
      | %<Vbase>V
      | %<VLF>pu
      | %<angleLF>deg.
      | %<Name>
  bus277 : powerlib/Measurements/Load Flow Bus  LConnTagsString=a  ID=bus277  Vbase=330000  Vref=1  Vangle=0  VLF=1  angleLF=0
      settings: AttributesFormatString=|
      | %<ID>
      | %<Vbase>V
      | %<VLF>pu
      | %<angleLF>deg.
      | %<Name>
  bus278 : powerlib/Measurements/Load Flow Bus  LConnTagsString=a  ID=bus278  Vbase=330000  Vref=1  Vangle=0  VLF=1  angleLF=0
      settings: AttributesFormatString=|
      | %<ID>
      | %<Vbase>V
      | %<VLF>pu
      | %<angleLF>deg.
      | %<Name>
  bus279 : powerlib/Measurements/Load Flow Bus  LConnTagsString=a  ID=bus279  Vbase=330000  Vref=1  Vangle=0  VLF=1  angleLF=0
      settings: AttributesFormatString=|
      | %<ID>
      | %<Vbase>V
      | %<VLF>pu
      | %<angleLF>deg.
      | %<Name>
  bus28 : powerlib/Measurements/Load Flow Bus  LConnTagsString=a  ID=bus28  Vbase=110000  Vref=1  Vangle=0  VLF=1  angleLF=0
      settings: AttributesFormatString=|
      | %<ID>
      | %<Vbase>V
      | %<VLF>pu
      | %<angleLF>deg.
      | %<Name>
  bus280 : powerlib/Measurements/Load Flow Bus  LConnTagsString=a  ID=bus280  Vbase=330000  Vref=1  Vangle=0  VLF=1  angleLF=0
      settings: AttributesFormatString=|
      | %<ID>
      | %<Vbase>V
      | %<VLF>pu
      | %<angleLF>deg.
      | %<Name>
  bus281 : powerlib/Measurements/Load Flow Bus  LConnTagsString=a  ID=bus281  Vbase=330000  Vref=1  Vangle=0  VLF=1  angleLF=0
      settings: AttributesFormatString=|
      | %<ID>
      | %<Vbase>V
      | %<VLF>pu
      | %<angleLF>deg.
      | %<Name>
  bus282 : powerlib/Measurements/Load Flow Bus  LConnTagsString=a  ID=bus282  Vbase=330000  Vref=1  Vangle=0  VLF=1  angleLF=0
      settings: AttributesFormatString=|
      | %<ID>
      | %<Vbase>V
      | %<VLF>pu
      | %<angleLF>deg.
      | %<Name>
  bus283 : powerlib/Measurements/Load Flow Bus  LConnTagsString=a  ID=bus283  Vbase=330000  Vref=1  Vangle=0  VLF=1  angleLF=0
      settings: AttributesFormatString=|
      | %<ID>
      | %<Vbase>V
      | %<VLF>pu
      | %<angleLF>deg.
      | %<Name>
  bus284 : powerlib/Measurements/Load Flow Bus  LConnTagsString=a  ID=bus284  Vbase=330000  Vref=1  Vangle=0  VLF=1  angleLF=0
      settings: AttributesFormatString=|
      | %<ID>
      | %<Vbase>V
      | %<VLF>pu
      | %<angleLF>deg.
      | %<Name>
  bus285 : powerlib/Measurements/Load Flow Bus  LConnTagsString=a  ID=bus285  Vbase=330000  Vref=1  Vangle=0  VLF=1  angleLF=0
      settings: AttributesFormatString=|
      | %<ID>
      | %<Vbase>V
      | %<VLF>pu
      | %<angleLF>deg.
      | %<Name>
  bus286 : powerlib/Measurements/Load Flow Bus  LConnTagsString=a  ID=bus286  Vbase=330000  Vref=1  Vangle=0  VLF=1  angleLF=0
      settings: AttributesFormatString=|
      | %<ID>
      | %<Vbase>V
      | %<VLF>pu
      | %<angleLF>deg.
      | %<Name>
  bus287 : powerlib/Measurements/Load Flow Bus  LConnTagsString=a  ID=bus287  Vbase=330000  Vref=1  Vangle=0  VLF=1  angleLF=0
      settings: AttributesFormatString=|
      | %<ID>
      | %<Vbase>V
      | %<VLF>pu
      | %<angleLF>deg.
      | %<Name>
  bus288 : powerlib/Measurements/Load Flow Bus  LConnTagsString=a  ID=bus288  Vbase=330000  Vref=1  Vangle=0  VLF=1  angleLF=0
      settings: AttributesFormatString=|
      | %<ID>
      | %<Vbase>V
      | %<VLF>pu
      | %<angleLF>deg.
      | %<Name>
  bus289 : powerlib/Measurements/Load Flow Bus  LConnTagsString=a  ID=bus289  Vbase=330000  Vref=1  Vangle=0  VLF=1  angleLF=0
      settings: AttributesFormatString=|
      | %<ID>
      | %<Vbase>V
      | %<VLF>pu
      | %<angleLF>deg.
      | %<Name>
  bus29 : powerlib/Measurements/Load Flow Bus  LConnTagsString=a  ID=bus29  Vbase=110000  Vref=1  Vangle=0  VLF=1  angleLF=0
      settings: AttributesFormatString=|
      | %<ID>
      | %<Vbase>V
      | %<VLF>pu
      | %<angleLF>deg.
      | %<Name>
  bus290 : powerlib/Measurements/Load Flow Bus  LConnTagsString=a  ID=bus290  Vbase=330000  Vref=1  Vangle=0  VLF=1  angleLF=0
      settings: AttributesFormatString=|
      | %<ID>
      | %<Vbase>V
      | %<VLF>pu
      | %<angleLF>deg.
      | %<Name>
  bus291 : powerlib/Measurements/Load Flow Bus  LConnTagsString=a  ID=bus291  Vbase=330000  Vref=1  Vangle=0  VLF=1  angleLF=0
      settings: AttributesFormatString=|
      | %<ID>
      | %<Vbase>V
      | %<VLF>pu
      | %<angleLF>deg.
      | %<Name>
  bus3 : powerlib/Measurements/Load Flow Bus  LConnTagsString=a  ID=bus3  Vbase=110000  Vref=1  Vangle=0  VLF=1  angleLF=0
      settings: AttributesFormatString=|
      | %<ID>
      | %<Vbase>V
      | %<VLF>pu
      | %<angleLF>deg.
      | %<Name>
  bus30 : powerlib/Measurements/Load Flow Bus  LConnTagsString=a  ID=bus30  Vbase=110000  Vref=1  Vangle=0  VLF=1  angleLF=0
      settings: AttributesFormatString=|
      | %<ID>
      | %<Vbase>V
      | %<VLF>pu
      | %<angleLF>deg.
      | %<Name>
  bus31 : powerlib/Measurements/Load Flow Bus  LConnTagsString=a  ID=bus31  Vbase=110000  Vref=1  Vangle=0  VLF=1  angleLF=0
      settings: AttributesFormatString=|
      | %<ID>
      | %<Vbase>V
      | %<VLF>pu
      | %<angleLF>deg.
      | %<Name>
  bus32 : powerlib/Measurements/Load Flow Bus  LConnTagsString=a  ID=bus32  Vbase=110000  Vref=1  Vangle=0  VLF=1  angleLF=0
      settings: AttributesFormatString=|
      | %<ID>
      | %<Vbase>V
      | %<VLF>pu
      | %<angleLF>deg.
      | %<Name>
  bus33 : powerlib/Measurements/Load Flow Bus  LConnTagsString=a  ID=bus33  Vbase=110000  Vref=1  Vangle=0  VLF=1  angleLF=0
      settings: AttributesFormatString=|
      | %<ID>
      | %<Vbase>V
      | %<VLF>pu
      | %<angleLF>deg.
      | %<Name>
  bus34 : powerlib/Measurements/Load Flow Bus  LConnTagsString=a  ID=bus34  Vbase=110000  Vref=1  Vangle=0  VLF=1  angleLF=0
      settings: AttributesFormatString=|
      | %<ID>
      | %<Vbase>V
      | %<VLF>pu
      | %<angleLF>deg.
      | %<Name>
  bus35 : powerlib/Measurements/Load Flow Bus  LConnTagsString=a  ID=bus35  Vbase=110000  Vref=1  Vangle=0  VLF=1  angleLF=0
      settings: AttributesFormatString=|
      | %<ID>
      | %<Vbase>V
      | %<VLF>pu
      | %<angleLF>deg.
      | %<Name>
  bus36 : powerlib/Measurements/Load Flow Bus  LConnTagsString=a  ID=bus36  Vbase=110000  Vref=1  Vangle=0  VLF=1  angleLF=0
      settings: AttributesFormatString=|
      | %<ID>
      | %<Vbase>V
      | %<VLF>pu
      | %<angleLF>deg.
      | %<Name>
  bus37 : powerlib/Measurements/Load Flow Bus  LConnTagsString=a  ID=bus37  Vbase=110000  Vref=1  Vangle=0  VLF=1  angleLF=0
      settings: AttributesFormatString=|
      | %<ID>
      | %<Vbase>V
      | %<VLF>pu
      | %<angleLF>deg.
      | %<Name>
  bus38 : powerlib/Measurements/Load Flow Bus  LConnTagsString=a  ID=bus38  Vbase=110000  Vref=1  Vangle=0  VLF=1  angleLF=0
      settings: AttributesFormatString=|
      | %<ID>
      | %<Vbase>V
      | %<VLF>pu
      | %<angleLF>deg.
      | %<Name>
  bus39 : powerlib/Measurements/Load Flow Bus  LConnTagsString=a  ID=bus39  Vbase=110000  Vref=1  Vangle=0  VLF=1  angleLF=0
      settings: AttributesFormatString=|
      | %<ID>
      | %<Vbase>V
      | %<VLF>pu
      | %<angleLF>deg.
      | %<Name>
  bus4 : powerlib/Measurements/Load Flow Bus  LConnTagsString=a  ID=bus4  Vbase=110000  Vref=1  Vangle=0  VLF=1  angleLF=0
      settings: AttributesFormatString=|
      | %<ID>
      | %<Vbase>V
      | %<VLF>pu
      | %<angleLF>deg.
      | %<Name>
  bus40 : powerlib/Measurements/Load Flow Bus  LConnTagsString=a  ID=bus40  Vbase=110000  Vref=1  Vangle=0  VLF=1  angleLF=0
      settings: AttributesFormatString=|
      | %<ID>
      | %<Vbase>V
      | %<VLF>pu
      | %<angleLF>deg.
      | %<Name>
  bus41 : powerlib/Measurements/Load Flow Bus  LConnTagsString=a  ID=bus41  Vbase=110000  Vref=1  Vangle=0  VLF=1  angleLF=0
      settings: AttributesFormatString=|
      | %<ID>
      | %<Vbase>V
      | %<VLF>pu
      | %<angleLF>deg.
      | %<Name>
  bus42 : powerlib/Measurements/Load Flow Bus  LConnTagsString=a  ID=bus42  Vbase=110000  Vref=1  Vangle=0  VLF=1  angleLF=0
      settings: AttributesFormatString=|
      | %<ID>
      | %<Vbase>V
      | %<VLF>pu
      | %<angleLF>deg.
      | %<Name>
  bus43 : powerlib/Measurements/Load Flow Bus  LConnTagsString=a  ID=bus43  Vbase=110000  Vref=1  Vangle=0  VLF=1  angleLF=0
      settings: AttributesFormatString=|
      | %<ID>
      | %<Vbase>V
      | %<VLF>pu
      | %<angleLF>deg.
      | %<Name>
  bus44 : powerlib/Measurements/Load Flow Bus  LConnTagsString=a  ID=bus44  Vbase=110000  Vref=1  Vangle=0  VLF=1  angleLF=0
      settings: AttributesFormatString=|
      | %<ID>
      | %<Vbase>V
      | %<VLF>pu
      | %<angleLF>deg.
      | %<Name>
  bus45 : powerlib/Measurements/Load Flow Bus  LConnTagsString=a  ID=bus45  Vbase=110000  Vref=1  Vangle=0  VLF=1  angleLF=0
      settings: AttributesFormatString=|
      | %<ID>
      | %<Vbase>V
      | %<VLF>pu
      | %<angleLF>deg.
      | %<Name>
  bus46 : powerlib/Measurements/Load Flow Bus  LConnTagsString=a  ID=bus46  Vbase=110000  Vref=1  Vangle=0  VLF=1  angleLF=0
      settings: AttributesFormatString=|
      | %<ID>
      | %<Vbase>V
      | %<VLF>pu
      | %<angleLF>deg.
      | %<Name>
  bus47 : powerlib/Measurements/Load Flow Bus  LConnTagsString=a  ID=bus47  Vbase=110000  Vref=1  Vangle=0  VLF=1  angleLF=0
      settings: AttributesFormatString=|
      | %<ID>
      | %<Vbase>V
      | %<VLF>pu
      | %<angleLF>deg.
      | %<Name>
  bus48 : powerlib/Measurements/Load Flow Bus  LConnTagsString=a  ID=bus48  Vbase=110000  Vref=1  Vangle=0  VLF=1  angleLF=0
      settings: AttributesFormatString=|
      | %<ID>
      | %<Vbase>V
      | %<VLF>pu
      | %<angleLF>deg.
      | %<Name>
  bus49 : powerlib/Measurements/Load Flow Bus  LConnTagsString=a  ID=bus49  Vbase=110000  Vref=1  Vangle=0  VLF=1  angleLF=0
      settings: AttributesFormatString=|
      | %<ID>
      | %<Vbase>V
      | %<VLF>pu
      | %<angleLF>deg.
      | %<Name>
  bus5 : powerlib/Measurements/Load Flow Bus  LConnTagsString=a  ID=bus5  Vbase=110000  Vref=1  Vangle=0  VLF=1  angleLF=0
      settings: AttributesFormatString=|
      | %<ID>
      | %<Vbase>V
      | %<VLF>pu
      | %<angleLF>deg.
      | %<Name>
  bus50 : powerlib/Measurements/Load Flow Bus  LConnTagsString=a  ID=bus50  Vbase=110000  Vref=1  Vangle=0  VLF=1  angleLF=0
      settings: AttributesFormatString=|
      | %<ID>
      | %<Vbase>V
      | %<VLF>pu
      | %<angleLF>deg.
      | %<Name>
  bus51 : powerlib/Measurements/Load Flow Bus  LConnTagsString=a  ID=bus51  Vbase=110000  Vref=1  Vangle=0  VLF=1  angleLF=0
      settings: AttributesFormatString=|
      | %<ID>
      | %<Vbase>V
      | %<VLF>pu
      | %<angleLF>deg.
      | %<Name>
  bus52 : powerlib/Measurements/Load Flow Bus  LConnTagsString=a  ID=bus52  Vbase=110000  Vref=1  Vangle=0  VLF=1  angleLF=0
      settings: AttributesFormatString=|
      | %<ID>
      | %<Vbase>V
      | %<VLF>pu
      | %<angleLF>deg.
      | %<Name>
  bus53 : powerlib/Measurements/Load Flow Bus  LConnTagsString=a  ID=bus53  Vbase=110000  Vref=1  Vangle=0  VLF=1  angleLF=0
      settings: AttributesFormatString=|
      | %<ID>
      | %<Vbase>V
      | %<VLF>pu
      | %<angleLF>deg.
      | %<Name>
  bus54 : powerlib/Measurements/Load Flow Bus  LConnTagsString=a  ID=bus54  Vbase=110000  Vref=1  Vangle=0  VLF=1  angleLF=0
      settings: AttributesFormatString=|
      | %<ID>
      | %<Vbase>V
      | %<VLF>pu
      | %<angleLF>deg.
      | %<Name>
  bus55 : powerlib/Measurements/Load Flow Bus  LConnTagsString=a  ID=bus55  Vbase=110000  Vref=1  Vangle=0  VLF=1  angleLF=0
      settings: AttributesFormatString=|
      | %<ID>
      | %<Vbase>V
      | %<VLF>pu
      | %<angleLF>deg.
      | %<Name>
  bus56 : powerlib/Measurements/Load Flow Bus  LConnTagsString=a  ID=bus56  Vbase=110000  Vref=1  Vangle=0  VLF=1  angleLF=0
      settings: AttributesFormatString=|
      | %<ID>
      | %<Vbase>V
      | %<VLF>pu
      | %<angleLF>deg.
      | %<Name>
  bus57 : powerlib/Measurements/Load Flow Bus  LConnTagsString=a  ID=bus57  Vbase=110000  Vref=1  Vangle=0  VLF=1  angleLF=0
      settings: AttributesFormatString=|
      | %<ID>
      | %<Vbase>V
      | %<VLF>pu
      | %<angleLF>deg.
      | %<Name>
  bus58 : powerlib/Measurements/Load Flow Bus  LConnTagsString=a  ID=bus58  Vbase=110000  Vref=1  Vangle=0  VLF=1  angleLF=0
      settings: AttributesFormatString=|
      | %<ID>
      | %<Vbase>V
      | %<VLF>pu
      | %<angleLF>deg.
      | %<Name>
  bus59 : powerlib/Measurements/Load Flow Bus  LConnTagsString=a  ID=bus59  Vbase=110000  Vref=1  Vangle=0  VLF=1  angleLF=0
      settings: AttributesFormatString=|
      | %<ID>
      | %<Vbase>V
      | %<VLF>pu
      | %<angleLF>deg.
      | %<Name>
  bus6 : powerlib/Measurements/Load Flow Bus  LConnTagsString=a  ID=bus6  Vbase=110000  Vref=1  Vangle=0  VLF=1  angleLF=0
      settings: AttributesFormatString=|
      | %<ID>
      | %<Vbase>V
      | %<VLF>pu
      | %<angleLF>deg.
      | %<Name>
  bus60 : powerlib/Measurements/Load Flow Bus  LConnTagsString=a  ID=bus60  Vbase=110000  Vref=1  Vangle=0  VLF=1  angleLF=0
      settings: AttributesFormatString=|
      | %<ID>
      | %<Vbase>V
      | %<VLF>pu
      | %<angleLF>deg.
      | %<Name>
  bus61 : powerlib/Measurements/Load Flow Bus  LConnTagsString=a  ID=bus61  Vbase=110000  Vref=1  Vangle=0  VLF=1  angleLF=0
      settings: AttributesFormatString=|
      | %<ID>
      | %<Vbase>V
      | %<VLF>pu
      | %<angleLF>deg.
      | %<Name>
  bus62 : powerlib/Measurements/Load Flow Bus  LConnTagsString=a  ID=bus62  Vbase=110000  Vref=1  Vangle=0  VLF=1  angleLF=0
      settings: AttributesFormatString=|
      | %<ID>
      | %<Vbase>V
      | %<VLF>pu
      | %<angleLF>deg.
      | %<Name>
  bus63 : powerlib/Measurements/Load Flow Bus  LConnTagsString=a  ID=bus63  Vbase=110000  Vref=1  Vangle=0  VLF=1  angleLF=0
      settings: AttributesFormatString=|
      | %<ID>
      | %<Vbase>V
      | %<VLF>pu
      | %<angleLF>deg.
      | %<Name>
  bus64 : powerlib/Measurements/Load Flow Bus  LConnTagsString=a  ID=bus64  Vbase=110000  Vref=1  Vangle=0  VLF=1  angleLF=0
      settings: AttributesFormatString=|
      | %<ID>
      | %<Vbase>V
      | %<VLF>pu
      | %<angleLF>deg.
      | %<Name>
  bus65 : powerlib/Measurements/Load Flow Bus  LConnTagsString=a  ID=bus65  Vbase=110000  Vref=1  Vangle=0  VLF=1  angleLF=0
      settings: AttributesFormatString=|
      | %<ID>
      | %<Vbase>V
      | %<VLF>pu
      | %<angleLF>deg.
      | %<Name>
  bus66 : powerlib/Measurements/Load Flow Bus  LConnTagsString=a  ID=bus66  Vbase=110000  Vref=1  Vangle=0  VLF=1  angleLF=0
      settings: AttributesFormatString=|
      | %<ID>
      | %<Vbase>V
      | %<VLF>pu
      | %<angleLF>deg.
      | %<Name>
  bus67 : powerlib/Measurements/Load Flow Bus  LConnTagsString=a  ID=bus67  Vbase=110000  Vref=1  Vangle=0  VLF=1  angleLF=0
      settings: AttributesFormatString=|
      | %<ID>
      | %<Vbase>V
      | %<VLF>pu
      | %<angleLF>deg.
      | %<Name>
  bus68 : powerlib/Measurements/Load Flow Bus  LConnTagsString=a  ID=bus68  Vbase=110000  Vref=1  Vangle=0  VLF=1  angleLF=0
      settings: AttributesFormatString=|
      | %<ID>
      | %<Vbase>V
      | %<VLF>pu
      | %<angleLF>deg.
      | %<Name>
  bus69 : powerlib/Measurements/Load Flow Bus  LConnTagsString=a  ID=bus69  Vbase=110000  Vref=1  Vangle=0  VLF=1  angleLF=0
      settings: AttributesFormatString=|
      | %<ID>
      | %<Vbase>V
      | %<VLF>pu
      | %<angleLF>deg.
      | %<Name>
  bus7 : powerlib/Measurements/Load Flow Bus  LConnTagsString=a  ID=bus7  Vbase=110000  Vref=1  Vangle=0  VLF=1  angleLF=0
      settings: AttributesFormatString=|
      | %<ID>
      | %<Vbase>V
      | %<VLF>pu
      | %<angleLF>deg.
      | %<Name>
  bus70 : powerlib/Measurements/Load Flow Bus  LConnTagsString=a  ID=bus70  Vbase=110000  Vref=1  Vangle=0  VLF=1  angleLF=0
      settings: AttributesFormatString=|
      | %<ID>
      | %<Vbase>V
      | %<VLF>pu
      | %<angleLF>deg.
      | %<Name>
  bus71 : powerlib/Measurements/Load Flow Bus  LConnTagsString=a  ID=bus71  Vbase=110000  Vref=1  Vangle=0  VLF=1  angleLF=0
      settings: AttributesFormatString=|
      | %<ID>
      | %<Vbase>V
      | %<VLF>pu
      | %<angleLF>deg.
      | %<Name>
  bus72 : powerlib/Measurements/Load Flow Bus  LConnTagsString=a  ID=bus72  Vbase=110000  Vref=1  Vangle=0  VLF=1  angleLF=0
      settings: AttributesFormatString=|
      | %<ID>
      | %<Vbase>V
      | %<VLF>pu
      | %<angleLF>deg.
      | %<Name>
  bus73 : powerlib/Measurements/Load Flow Bus  LConnTagsString=a  ID=bus73  Vbase=110000  Vref=1  Vangle=0  VLF=1  angleLF=0
      settings: AttributesFormatString=|
      | %<ID>
      | %<Vbase>V
      | %<VLF>pu
      | %<angleLF>deg.
      | %<Name>
  bus74 : powerlib/Measurements/Load Flow Bus  LConnTagsString=a  ID=bus74  Vbase=110000  Vref=1  Vangle=0  VLF=1  angleLF=0
      settings: AttributesFormatString=|
      | %<ID>
      | %<Vbase>V
      | %<VLF>pu
      | %<angleLF>deg.
      | %<Name>
  bus75 : powerlib/Measurements/Load Flow Bus  LConnTagsString=a  ID=bus75  Vbase=110000  Vref=1  Vangle=0  VLF=1  angleLF=0
      settings: AttributesFormatString=|
      | %<ID>
      | %<Vbase>V
      | %<VLF>pu
      | %<angleLF>deg.
      | %<Name>
  bus76 : powerlib/Measurements/Load Flow Bus  LConnTagsString=a  ID=bus76  Vbase=110000  Vref=1  Vangle=0  VLF=1  angleLF=0
      settings: AttributesFormatString=|
      | %<ID>
      | %<Vbase>V
      | %<VLF>pu
      | %<angleLF>deg.
      | %<Name>
  bus77 : powerlib/Measurements/Load Flow Bus  LConnTagsString=a  ID=bus77  Vbase=110000  Vref=1  Vangle=0  VLF=1  angleLF=0
      settings: AttributesFormatString=|
      | %<ID>
      | %<Vbase>V
      | %<VLF>pu
      | %<angleLF>deg.
      | %<Name>
  bus78 : powerlib/Measurements/Load Flow Bus  LConnTagsString=a  ID=bus78  Vbase=110000  Vref=1  Vangle=0  VLF=1  angleLF=0
      settings: AttributesFormatString=|
      | %<ID>
      | %<Vbase>V
      | %<VLF>pu
      | %<angleLF>deg.
      | %<Name>
  bus79 : powerlib/Measurements/Load Flow Bus  LConnTagsString=a  ID=bus79  Vbase=110000  Vref=1  Vangle=0  VLF=1  angleLF=0
      settings: AttributesFormatString=|
      | %<ID>
      | %<Vbase>V
      | %<VLF>pu
      | %<angleLF>deg.
      | %<Name>
  bus8 : powerlib/Measurements/Load Flow Bus  LConnTagsString=a  ID=bus8  Vbase=110000  Vref=1  Vangle=0  VLF=1  angleLF=0
      settings: AttributesFormatString=|
      | %<ID>
      | %<Vbase>V
      | %<VLF>pu
      | %<angleLF>deg.
      | %<Name>
  bus80 : powerlib/Measurements/Load Flow Bus  LConnTagsString=a  ID=bus80  Vbase=110000  Vref=1  Vangle=0  VLF=1  angleLF=0
      settings: AttributesFormatString=|
      | %<ID>
      | %<Vbase>V
      | %<VLF>pu
      | %<angleLF>deg.
      | %<Name>
  bus81 : powerlib/Measurements/Load Flow Bus  LConnTagsString=a  ID=bus81  Vbase=110000  Vref=1  Vangle=0  VLF=1  angleLF=0
      settings: AttributesFormatString=|
      | %<ID>
      | %<Vbase>V
      | %<VLF>pu
      | %<angleLF>deg.
      | %<Name>
  bus82 : powerlib/Measurements/Load Flow Bus  LConnTagsString=a  ID=bus82  Vbase=110000  Vref=1  Vangle=0  VLF=1  angleLF=0
      settings: AttributesFormatString=|
      | %<ID>
      | %<Vbase>V
      | %<VLF>pu
      | %<angleLF>deg.
      | %<Name>
  bus83 : powerlib/Measurements/Load Flow Bus  LConnTagsString=a  ID=bus83  Vbase=110000  Vref=1  Vangle=0  VLF=1  angleLF=0
      settings: AttributesFormatString=|
      | %<ID>
      | %<Vbase>V
      | %<VLF>pu
      | %<angleLF>deg.
      | %<Name>
  bus84 : powerlib/Measurements/Load Flow Bus  LConnTagsString=a  ID=bus84  Vbase=110000  Vref=1  Vangle=0  VLF=1  angleLF=0
      settings: AttributesFormatString=|
      | %<ID>
      | %<Vbase>V
      | %<VLF>pu
      | %<angleLF>deg.
      | %<Name>
  bus85 : powerlib/Measurements/Load Flow Bus  LConnTagsString=a  ID=bus85  Vbase=110000  Vref=1  Vangle=0  VLF=1  angleLF=0
      settings: AttributesFormatString=|
      | %<ID>
      | %<Vbase>V
      | %<VLF>pu
      | %<angleLF>deg.
      | %<Name>
  bus86 : powerlib/Measurements/Load Flow Bus  LConnTagsString=a  ID=bus86  Vbase=110000  Vref=1  Vangle=0  VLF=1  angleLF=0
      settings: AttributesFormatString=|
      | %<ID>
      | %<Vbase>V
      | %<VLF>pu
      | %<angleLF>deg.
      | %<Name>
  bus87 : powerlib/Measurements/Load Flow Bus  LConnTagsString=a  ID=bus87  Vbase=110000  Vref=1  Vangle=0  VLF=1  angleLF=0
      settings: AttributesFormatString=|
      | %<ID>
      | %<Vbase>V
      | %<VLF>pu
      | %<angleLF>deg.
      | %<Name>
  bus88 : powerlib/Measurements/Load Flow Bus  LConnTagsString=a  ID=bus88  Vbase=110000  Vref=1  Vangle=0  VLF=1  angleLF=0
      settings: AttributesFormatString=|
      | %<ID>
      | %<Vbase>V
      | %<VLF>pu
      | %<angleLF>deg.
      | %<Name>
  bus89 : powerlib/Measurements/Load Flow Bus  LConnTagsString=a  ID=bus89  Vbase=110000  Vref=1  Vangle=0  VLF=1  angleLF=0
      settings: AttributesFormatString=|
      | %<ID>
      | %<Vbase>V
      | %<VLF>pu
      | %<angleLF>deg.
      | %<Name>
  bus9 : powerlib/Measurements/Load Flow Bus  LConnTagsString=a  ID=bus9  Vbase=110000  Vref=1  Vangle=0  VLF=1  angleLF=0
      settings: AttributesFormatString=|
      | %<ID>
      | %<Vbase>V
      | %<VLF>pu
      | %<angleLF>deg.
      | %<Name>
  bus90 : powerlib/Measurements/Load Flow Bus  LConnTagsString=a  ID=bus90  Vbase=110000  Vref=1  Vangle=0  VLF=1  angleLF=0
      settings: AttributesFormatString=|
      | %<ID>
      | %<Vbase>V
      | %<VLF>pu
      | %<angleLF>deg.
      | %<Name>
  bus91 : powerlib/Measurements/Load Flow Bus  LConnTagsString=a  ID=bus91  Vbase=110000  Vref=1  Vangle=0  VLF=1  angleLF=0
      settings: AttributesFormatString=|
      | %<ID>
      | %<Vbase>V
      | %<VLF>pu
      | %<angleLF>deg.
      | %<Name>
  bus92 : powerlib/Measurements/Load Flow Bus  LConnTagsString=a  ID=bus92  Vbase=110000  Vref=1  Vangle=0  VLF=1  angleLF=0
      settings: AttributesFormatString=|
      | %<ID>
      | %<Vbase>V
      | %<VLF>pu
      | %<angleLF>deg.
      | %<Name>
  bus93 : powerlib/Measurements/Load Flow Bus  LConnTagsString=a  ID=bus93  Vbase=110000  Vref=1  Vangle=0  VLF=1  angleLF=0
      settings: AttributesFormatString=|
      | %<ID>
      | %<Vbase>V
      | %<VLF>pu
      | %<angleLF>deg.
      | %<Name>
  bus94 : powerlib/Measurements/Load Flow Bus  LConnTagsString=a  ID=bus94  Vbase=110000  Vref=1  Vangle=0  VLF=1  angleLF=0
      settings: AttributesFormatString=|
      | %<ID>
      | %<Vbase>V
      | %<VLF>pu
      | %<angleLF>deg.
      | %<Name>
  bus95 : powerlib/Measurements/Load Flow Bus  LConnTagsString=a  ID=bus95  Vbase=110000  Vref=1  Vangle=0  VLF=1  angleLF=0
      settings: AttributesFormatString=|
      | %<ID>
      | %<Vbase>V
      | %<VLF>pu
      | %<angleLF>deg.
      | %<Name>
  bus96 : powerlib/Measurements/Load Flow Bus  LConnTagsString=a  ID=bus96  Vbase=110000  Vref=1  Vangle=0  VLF=1  angleLF=0
      settings: AttributesFormatString=|
      | %<ID>
      | %<Vbase>V
      | %<VLF>pu
      | %<angleLF>deg.
      | %<Name>
  bus97 : powerlib/Measurements/Load Flow Bus  LConnTagsString=a  ID=bus97  Vbase=110000  Vref=1  Vangle=0  VLF=1  angleLF=0
      settings: AttributesFormatString=|
      | %<ID>
      | %<Vbase>V
      | %<VLF>pu
      | %<angleLF>deg.
      | %<Name>
  bus98 : powerlib/Measurements/Load Flow Bus  LConnTagsString=a  ID=bus98  Vbase=110000  Vref=1  Vangle=0  VLF=1  angleLF=0
      settings: AttributesFormatString=|
      | %<ID>
      | %<Vbase>V
      | %<VLF>pu
      | %<angleLF>deg.
      | %<Name>
  bus99 : powerlib/Measurements/Load Flow Bus  LConnTagsString=a  ID=bus99  Vbase=110000  Vref=1  Vangle=0  VLF=1  angleLF=0
      settings: AttributesFormatString=|
      | %<ID>
      | %<Vbase>V
      | %<VLF>pu
      | %<angleLF>deg.
      | %<Name>
  powergui : powerlib/powergui  Priority=1  SimulationMode=Continuous  SolverType=Tustin  SampleTime=50e-6  frequency=60  SPID=off  DisableSnubberDevices=off  DisableRonSwitches=off  DisableVfSwitches=off  SwTol=0  Interpol=off  DisplayEquations=off  Ts=0  methode=off  frequencyindice=60  Pbase=100e6  ErrMax=1e-4  Iterations=50  UnitsV=kV  UnitsW=MW  FunctionMessages=off  echomessages=off  HookPort=off  EnableUseOfTLC=off  x0status=blocks  RestoreLinks=warning  ResistiveCurrentMeasurement=off  Frange=[0:2:500]  Ylog=off  Xlog=on  ShowGrid=off  save=off  variable=ZData  structure=0  ZoomFFT=off  StartTime=0.0  cycles=1  DisplayStyle=1  fundamental=60  FreqAxis=off  MaxFrequency=1000  frequencyindicesteady=1  RmsSteady=1  display=off
  ВЛ_220_кВ_Инта___Воркута_CN_177805996_220000_CN_88433653_220000 : powerlib/Elements/Distributed Parameters Line  Phases=3  Frequency=60  Resistance=[0.01273 0.3864]  Inductance="[0.9337e-3  4.1264e-3]"  Capacitance=[12.74e-9 7.751e-9]  Length=38.5055  x1=[0 0 0 0; 0.0001244 0 0 0; 0.0002488 0 0 0; 0.0003733 0 0 0; 0.0004977 0 0 0; 0.0006221 0 0 0]  x2=[0 0 0 0; 0.0001244 0 0 0; 0.0002488 0 0 0; 0.0003733 0 0 0; 0.0004977 0 0 0; 0.0006221 0 0 0]  x3=[0 0 0 0; 0.0001244 0 0 0; 0.0002488 0 0 0; 0.0003733 0 0 0; 0.0004977 0 0 0; 0.0006221 0 0 0]  x4=[0 0 0 0; 0.0001244 0 0 0; 0.0002488 0 0 0; 0.0003733 0 0 0; 0.0004977 0 0 0; 0.0006221 0 0 0]  x5=0  V1=ones(3,3)  V2=ones(3,3)  I1=ones(3,3)  I2=ones(3,3)  nHarmo=1  Measurements=None
  Вельск___Шангалы_CN_147416198_220000_CN_265498319_220000 : powerlib/Elements/Distributed Parameters Line  Phases=3  Frequency=60  Resistance=[0.01273 0.3864]  Inductance="[0.9337e-3  4.1264e-3]"  Capacitance=[12.74e-9 7.751e-9]  Length=78.8407  x1=[0 0 0 0; 0.0001244 0 0 0; 0.0002488 0 0 0; 0.0003733 0 0 0; 0.0004977 0 0 0; 0.0006221 0 0 0]  x2=[0 0 0 0; 0.0001244 0 0 0; 0.0002488 0 0 0; 0.0003733 0 0 0; 0.0004977 0 0 0; 0.0006221 0 0 0]  x3=[0 0 0 0; 0.0001244 0 0 0; 0.0002488 0 0 0; 0.0003733 0 0 0; 0.0004977 0 0 0; 0.0006221 0 0 0]  x4=[0 0 0 0; 0.0001244 0 0 0; 0.0002488 0 0 0; 0.0003733 0 0 0; 0.0004977 0 0 0; 0.0006221 0 0 0]  x5=0  V1=ones(3,3)  V2=ones(3,3)  I1=ones(3,3)  I2=ones(3,3)  nHarmo=1  Measurements=None
  Заовражье___Кизема_CN_163253148_220000_CN_159848384_220000 : powerlib/Elements/Distributed Parameters Line  Phases=3  Frequency=60  Resistance=[0.01273 0.3864]  Inductance="[0.9337e-3  4.1264e-3]"  Capacitance=[12.74e-9 7.751e-9]  Length=92.1738  x1=[0 0 0 0; 0.0001244 0 0 0; 0.0002488 0 0 0; 0.0003733 0 0 0; 0.0004977 0 0 0; 0.0006221 0 0 0]  x2=[0 0 0 0; 0.0001244 0 0 0; 0.0002488 0 0 0; 0.0003733 0 0 0; 0.0004977 0 0 0; 0.0006221 0 0 0]  x3=[0 0 0 0; 0.0001244 0 0 0; 0.0002488 0 0 0; 0.0003733 0 0 0; 0.0004977 0 0 0; 0.0006221 0 0 0]  x4=[0 0 0 0; 0.0001244 0 0 0; 0.0002488 0 0 0; 0.0003733 0 0 0; 0.0004977 0 0 0; 0.0006221 0 0 0]  x5=0  V1=ones(3,3)  V2=ones(3,3)  I1=ones(3,3)  I2=ones(3,3)  nHarmo=1  Measurements=None
  Калининградская_ТЭЦ_2_–_ПС_О_1_«Центральная»_CN_296188566_330000_CN_302938336_330000 : powerlib/Elements/Distributed Parameters Line  Phases=3  Frequency=60  Resistance=[0.01273 0.3864]  Inductance="[0.9337e-3  4.1264e-3]"  Capacitance=[12.74e-9 7.751e-9]  Length=18.1279  x1=[0 0 0 0; 0.0001244 0 0 0; 0.0002488 0 0 0; 0.0003733 0 0 0; 0.0004977 0 0 0; 0.0006221 0 0 0]  x2=[0 0 0 0; 0.0001244 0 0 0; 0.0002488 0 0 0; 0.0003733 0 0 0; 0.0004977 0 0 0; 0.0006221 0 0 0]  x3=[0 0 0 0; 0.0001244 0 0 0; 0.0002488 0 0 0; 0.0003733 0 0 0; 0.0004977 0 0 0; 0.0006221 0 0 0]  x4=[0 0 0 0; 0.0001244 0 0 0; 0.0002488 0 0 0; 0.0003733 0 0 0; 0.0004977 0 0 0; 0.0006221 0 0 0]  x5=0  V1=ones(3,3)  V2=ones(3,3)  I1=ones(3,3)  I2=ones(3,3)  nHarmo=1  Measurements=None
  Калининградская_ТЭЦ_2_—_ПC_«Северная_330»_CN_296188566_330000_CN_53126382_330000 : powerlib/Elements/Distributed Parameters Line  Phases=3  Frequency=60  Resistance=[0.01273 0.3864]  Inductance="[0.9337e-3  4.1264e-3]"  Capacitance=[12.74e-9 7.751e-9]  Length=32.5032  x1=[0 0 0 0; 0.0001244 0 0 0; 0.0002488 0 0 0; 0.0003733 0 0 0; 0.0004977 0 0 0; 0.0006221 0 0 0]  x2=[0 0 0 0; 0.0001244 0 0 0; 0.0002488 0 0 0; 0.0003733 0 0 0; 0.0004977 0 0 0; 0.0006221 0 0 0]  x3=[0 0 0 0; 0.0001244 0 0 0; 0.0002488 0 0 0; 0.0003733 0 0 0; 0.0004977 0 0 0; 0.0006221 0 0 0]  x4=[0 0 0 0; 0.0001244 0 0 0; 0.0002488 0 0 0; 0.0003733 0 0 0; 0.0004977 0 0 0; 0.0006221 0 0 0]  x5=0  V1=ones(3,3)  V2=ones(3,3)  I1=ones(3,3)  I2=ones(3,3)  nHarmo=1  Measurements=None
  Кизема__Шангалы_CN_163253148_220000_CN_265498319_220000 : powerlib/Elements/Distributed Parameters Line  Phases=3  Frequency=60  Resistance=[0.01273 0.3864]  Inductance="[0.9337e-3  4.1264e-3]"  Capacitance=[12.74e-9 7.751e-9]  Length=38.9789  x1=[0 0 0 0; 0.0001244 0 0 0; 0.0002488 0 0 0; 0.0003733 0 0 0; 0.0004977 0 0 0; 0.0006221 0 0 0]  x2=[0 0 0 0; 0.0001244 0 0 0; 0.0002488 0 0 0; 0.0003733 0 0 0; 0.0004977 0 0 0; 0.0006221 0 0 0]  x3=[0 0 0 0; 0.0001244 0 0 0; 0.0002488 0 0 0; 0.0003733 0 0 0; 0.0004977 0 0 0; 0.0006221 0 0 0]  x4=[0 0 0 0; 0.0001244 0 0 0; 0.0002488 0 0 0; 0.0003733 0 0 0; 0.0004977 0 0 0; 0.0006221 0 0 0]  x5=0  V1=ones(3,3)  V2=ones(3,3)  I1=ones(3,3)  I2=ones(3,3)  nHarmo=1  Measurements=None
  Микунь___Сыктывкар_CN_217498367_220000_CN_211036038_220000 : powerlib/Elements/Distributed Parameters Line  Phases=3  Frequency=60  Resistance=[0.01273 0.3864]  Inductance="[0.9337e-3  4.1264e-3]"  Capacitance=[12.74e-9 7.751e-9]  Length=87.5372  x1=[0 0 0 0; 0.0001244 0 0 0; 0.0002488 0 0 0; 0.0003733 0 0 0; 0.0004977 0 0 0; 0.0006221 0 0 0]  x2=[0 0 0 0; 0.0001244 0 0 0; 0.0002488 0 0 0; 0.0003733 0 0 0; 0.0004977 0 0 0; 0.0006221 0 0 0]  x3=[0 0 0 0; 0.0001244 0 0 0; 0.0002488 0 0 0; 0.0003733 0 0 0; 0.0004977 0 0 0; 0.0006221 0 0 0]  x4=[0 0 0 0; 0.0001244 0 0 0; 0.0002488 0 0 0; 0.0003733 0 0 0; 0.0004977 0 0 0; 0.0006221 0 0 0]  x5=0  V1=ones(3,3)  V2=ones(3,3)  I1=ones(3,3)  I2=ones(3,3)  nHarmo=1  Measurements=None
  Плесецк___Новая_2_цепь_CN_163640749_220000_CN_124601500_220000 : powerlib/Elements/Distributed Parameters Line  Phases=3  Frequency=60  Resistance=[0.01273 0.3864]  Inductance="[0.9337e-3  4.1264e-3]"  Capacitance=[12.74e-9 7.751e-9]  Length=37.4192  x1=[0 0 0 0; 0.0001244 0 0 0; 0.0002488 0 0 0; 0.0003733 0 0 0; 0.0004977 0 0 0; 0.0006221 0 0 0]  x2=[0 0 0 0; 0.0001244 0 0 0; 0.0002488 0 0 0; 0.0003733 0 0 0; 0.0004977 0 0 0; 0.0006221 0 0 0]  x3=[0 0 0 0; 0.0001244 0 0 0; 0.0002488 0 0 0; 0.0003733 0 0 0; 0.0004977 0 0 0; 0.0006221 0 0 0]  x4=[0 0 0 0; 0.0001244 0 0 0; 0.0002488 0 0 0; 0.0003733 0 0 0; 0.0004977 0 0 0; 0.0006221 0 0 0]  x5=0  V1=ones(3,3)  V2=ones(3,3)  I1=ones(3,3)  I2=ones(3,3)  nHarmo=1  Measurements=None
  Синдор___Микунь_CN_212471066_220000_CN_211036038_220000 : powerlib/Elements/Distributed Parameters Line  Phases=3  Frequency=60  Resistance=[0.01273 0.3864]  Inductance="[0.9337e-3  4.1264e-3]"  Capacitance=[12.74e-9 7.751e-9]  Length=51.5065  x1=[0 0 0 0; 0.0001244 0 0 0; 0.0002488 0 0 0; 0.0003733 0 0 0; 0.0004977 0 0 0; 0.0006221 0 0 0]  x2=[0 0 0 0; 0.0001244 0 0 0; 0.0002488 0 0 0; 0.0003733 0 0 0; 0.0004977 0 0 0; 0.0006221 0 0 0]  x3=[0 0 0 0; 0.0001244 0 0 0; 0.0002488 0 0 0; 0.0003733 0 0 0; 0.0004977 0 0 0; 0.0006221 0 0 0]  x4=[0 0 0 0; 0.0001244 0 0 0; 0.0002488 0 0 0; 0.0003733 0 0 0; 0.0004977 0 0 0; 0.0006221 0 0 0]  x5=0  V1=ones(3,3)  V2=ones(3,3)  I1=ones(3,3)  I2=ones(3,3)  nHarmo=1  Measurements=None
  Усинская___Возейская_CN_105528914_220000_CN_260124523_220000 : powerlib/Elements/Distributed Parameters Line  Phases=3  Frequency=60  Resistance=[0.01273 0.3864]  Inductance="[0.9337e-3  4.1264e-3]"  Capacitance=[12.74e-9 7.751e-9]  Length=49.973  x1=[0 0 0 0; 0.0001244 0 0 0; 0.0002488 0 0 0; 0.0003733 0 0 0; 0.0004977 0 0 0; 0.0006221 0 0 0]  x2=[0 0 0 0; 0.0001244 0 0 0; 0.0002488 0 0 0; 0.0003733 0 0 0; 0.0004977 0 0 0; 0.0006221 0 0 0]  x3=[0 0 0 0; 0.0001244 0 0 0; 0.0002488 0 0 0; 0.0003733 0 0 0; 0.0004977 0 0 0; 0.0006221 0 0 0]  x4=[0 0 0 0; 0.0001244 0 0 0; 0.0002488 0 0 0; 0.0003733 0 0 0; 0.0004977 0 0 0; 0.0006221 0 0 0]  x5=0  V1=ones(3,3)  V2=ones(3,3)  I1=ones(3,3)  I2=ones(3,3)  nHarmo=1  Measurements=None
  Усинская___КС_УГПЗ_CN_105528914_220000_CN_331932782_220000 : powerlib/Elements/Distributed Parameters Line  Phases=3  Frequency=60  Resistance=[0.01273 0.3864]  Inductance="[0.9337e-3  4.1264e-3]"  Capacitance=[12.74e-9 7.751e-9]  Length=1.2878  x1=[0 0 0 0; 0.0001244 0 0 0; 0.0002488 0 0 0; 0.0003733 0 0 0; 0.0004977 0 0 0; 0.0006221 0 0 0]  x2=[0 0 0 0; 0.0001244 0 0 0; 0.0002488 0 0 0; 0.0003733 0 0 0; 0.0004977 0 0 0; 0.0006221 0 0 0]  x3=[0 0 0 0; 0.0001244 0 0 0; 0.0002488 0 0 0; 0.0003733 0 0 0; 0.0004977 0 0 0; 0.0006221 0 0 0]  x4=[0 0 0 0; 0.0001244 0 0 0; 0.0002488 0 0 0; 0.0003733 0 0 0; 0.0004977 0 0 0; 0.0006221 0 0 0]  x5=0  V1=ones(3,3)  V2=ones(3,3)  I1=ones(3,3)  I2=ones(3,3)  nHarmo=1  Measurements=None
  Усинская___Промысловая_CN_105535524_220000_CN_105528914_220000 : powerlib/Elements/Distributed Parameters Line  Phases=3  Frequency=60  Resistance=[0.01273 0.3864]  Inductance="[0.9337e-3  4.1264e-3]"  Capacitance=[12.74e-9 7.751e-9]  Length=4.2001  x1=[0 0 0 0; 0.0001244 0 0 0; 0.0002488 0 0 0; 0.0003733 0 0 0; 0.0004977 0 0 0; 0.0006221 0 0 0]  x2=[0 0 0 0; 0.0001244 0 0 0; 0.0002488 0 0 0; 0.0003733 0 0 0; 0.0004977 0 0 0; 0.0006221 0 0 0]  x3=[0 0 0 0; 0.0001244 0 0 0; 0.0002488 0 0 0; 0.0003733 0 0 0; 0.0004977 0 0 0; 0.0006221 0 0 0]  x4=[0 0 0 0; 0.0001244 0 0 0; 0.0002488 0 0 0; 0.0003733 0 0 0; 0.0004977 0 0 0; 0.0006221 0 0 0]  x5=0  V1=ones(3,3)  V2=ones(3,3)  I1=ones(3,3)  I2=ones(3,3)  nHarmo=1  Measurements=None
  Ухта___Синдор_CN_152126979_220000_CN_212471066_220000 : powerlib/Elements/Distributed Parameters Line  Phases=3  Frequency=60  Resistance=[0.01273 0.3864]  Inductance="[0.9337e-3  4.1264e-3]"  Capacitance=[12.74e-9 7.751e-9]  Length=106.1701  x1=[0 0 0 0; 0.0001244 0 0 0; 0.0002488 0 0 0; 0.0003733 0 0 0; 0.0004977 0 0 0; 0.0006221 0 0 0]  x2=[0 0 0 0; 0.0001244 0 0 0; 0.0002488 0 0 0; 0.0003733 0 0 0; 0.0004977 0 0 0; 0.0006221 0 0 0]  x3=[0 0 0 0; 0.0001244 0 0 0; 0.0002488 0 0 0; 0.0003733 0 0 0; 0.0004977 0 0 0; 0.0006221 0 0 0]  x4=[0 0 0 0; 0.0001244 0 0 0; 0.0002488 0 0 0; 0.0003733 0 0 0; 0.0004977 0 0 0; 0.0006221 0 0 0]  x5=0  V1=ones(3,3)  V2=ones(3,3)  I1=ones(3,3)  I2=ones(3,3)  nHarmo=1  Measurements=None
  connections:
  T_176029697__/LConn1 -- _CN_176029697_110000_CN_169809022_110000/LConn1
  T_176029697__/LConn2 -- _CN_176029697_110000_CN_169809022_110000/LConn2
  _CN_176029697_110000_CN_169809022_110000/LConn3 -- T_176029697__/LConn3 -- bus1/LConn1
  _CN_176029697_110000_CN_169809022_110000/RConn1 -- T_169809022__/RConn1 -- L_169809022/LConn1
  _CN_176029697_110000_CN_169809022_110000/RConn2 -- T_169809022__/RConn2 -- L_169809022/LConn2
  _CN_176029697_110000_CN_169809022_110000/RConn3 -- T_169809022__/RConn3 -- L_169809022/LConn3 -- bus2/LConn1
  T_279726507__ЭЧП_3/LConn1 -- _CN_279726507_110000_CN_144555400_110000/LConn1
  T_279726507__ЭЧП_3/LConn2 -- _CN_279726507_110000_CN_144555400_110000/LConn2
  _CN_279726507_110000_CN_144555400_110000/LConn3 -- T_279726507__ЭЧП_3/LConn3 -- bus3/LConn1
  T_144555400__ЭЧП_5/LConn1 -- _CN_279726507_110000_CN_144555400_110000/RConn1
  T_144555400__ЭЧП_5/LConn2 -- _CN_279726507_110000_CN_144555400_110000/RConn2
  _CN_279726507_110000_CN_144555400_110000/RConn3 -- T_144555400__ЭЧП_5/LConn3 -- bus4/LConn1
  T_184388878__Электростанция/LConn1 -- _CN_184388878_110000_CN_200446426_110000/LConn1
  T_184388878__Электростанция/LConn2 -- _CN_184388878_110000_CN_200446426_110000/LConn2
  _CN_184388878_110000_CN_200446426_110000/LConn3 -- T_184388878__Электростанция/LConn3 -- bus5/LConn1
  T_200446426__/LConn1 -- _CN_184388878_110000_CN_200446426_110000/RConn1
  T_200446426__/LConn2 -- _CN_184388878_110000_CN_200446426_110000/RConn2
  _CN_184388878_110000_CN_200446426_110000/RConn3 -- T_200446426__/LConn3 -- bus6/LConn1
  T_128423956__ЭПС_Мостищи_110_10_кВ/LConn1 -- _CN_128423956_110000_CN_184189206_110000/LConn1
  T_128423956__ЭПС_Мостищи_110_10_кВ/LConn2 -- _CN_128423956_110000_CN_184189206_110000/LConn2
  _CN_128423956_110000_CN_184189206_110000/LConn3 -- T_128423956__ЭПС_Мостищи_110_10_кВ/LConn3 -- bus7/LConn1
  T_184189206__ЭПС_Базовая:_110_10_6_кВ/LConn1 -- _CN_128423956_110000_CN_184189206_110000/RConn1
  T_184189206__ЭПС_Базовая:_110_10_6_кВ/LConn2 -- _CN_128423956_110000_CN_184189206_110000/RConn2
  _CN_128423956_110000_CN_184189206_110000/RConn3 -- T_184189206__ЭПС_Базовая:_110_10_6_кВ/LConn3 -- bus8/LConn1
  T_162611222__/LConn1 -- _CN_162611222_110000_CN_164224743_110000/LConn1
  T_162611222__/LConn2 -- _CN_162611222_110000_CN_164224743_110000/LConn2
  _CN_162611222_110000_CN_164224743_110000/LConn3 -- T_162611222__/LConn3 -- bus9/LConn1
  T_164224743__/LConn1 -- _CN_162611222_110000_CN_164224743_110000/RConn1
  T_164224743__/LConn2 -- _CN_162611222_110000_CN_164224743_110000/RConn2
  _CN_162611222_110000_CN_164224743_110000/RConn3 -- T_164224743__/LConn3 -- bus10/LConn1
  _CN_139107864_110000_CN_125823925_110000/LConn1 -- "T_139107864__Подстанция_\"Кораблестроительный_институт\""/LConn1 -- _CN_139107864_110000_CN_87108350_110000/LConn1
  _CN_139107864_110000_CN_125823925_110000/LConn2 -- "T_139107864__Подстанция_\"Кораблестроительный_институт\""/LConn2 -- _CN_139107864_110000_CN_87108350_110000/LConn2
  _CN_139107864_110000_CN_125823925_110000/LConn3 -- "T_139107864__Подстанция_\"Кораблестроительный_институт\""/LConn3 -- _CN_139107864_110000_CN_87108350_110000/LConn3 -- bus11/LConn1
  _CN_139107864_110000_CN_125823925_110000/RConn1 -- "T_125823925_330000_Подстация_\"Западная\""/RConn1 -- L_125823925/LConn1
  _CN_139107864_110000_CN_125823925_110000/RConn2 -- "T_125823925_330000_Подстация_\"Западная\""/RConn2 -- L_125823925/LConn2
  _CN_139107864_110000_CN_125823925_110000/RConn3 -- "T_125823925_330000_Подстация_\"Западная\""/RConn3 -- L_125823925/LConn3 -- bus12/LConn1
  T_87108350__/LConn1 -- _CN_139107864_110000_CN_87108350_110000/RConn1
  T_87108350__/LConn2 -- _CN_139107864_110000_CN_87108350_110000/RConn2
  _CN_139107864_110000_CN_87108350_110000/RConn3 -- T_87108350__/LConn3 -- bus13/LConn1
  _CN_160499737_110000_CN_114315616_110000/LConn1 -- "T_160499737_110000;10000_ПС_399_\"ЭТЗ_Псков\"_110_10_кВ"/LConn1 -- _CN_160499737_110000_CN_135051666_110000/LConn1 -- _CN_160499737_110000_CN_201631424_110000/LConn1
  _CN_160499737_110000_CN_114315616_110000/LConn2 -- "T_160499737_110000;10000_ПС_399_\"ЭТЗ_Псков\"_110_10_кВ"/LConn2 -- _CN_160499737_110000_CN_135051666_110000/LConn2 -- _CN_160499737_110000_CN_201631424_110000/LConn2
  _CN_160499737_110000_CN_114315616_110000/LConn3 -- "T_160499737_110000;10000_ПС_399_\"ЭТЗ_Псков\"_110_10_кВ"/LConn3 -- _CN_160499737_110000_CN_135051666_110000/LConn3 -- _CN_160499737_110000_CN_201631424_110000/LConn3 -- bus14/LConn1
  "T_114315616_110000;10000;6000_ПС_328_\"Заводская\"_110_10_6_кВ"/LConn1 -- _CN_160499737_110000_CN_114315616_110000/RConn1
  "T_114315616_110000;10000;6000_ПС_328_\"Заводская\"_110_10_6_кВ"/LConn2 -- _CN_160499737_110000_CN_114315616_110000/RConn2
  _CN_160499737_110000_CN_114315616_110000/RConn3 -- "T_114315616_110000;10000;6000_ПС_328_\"Заводская\"_110_10_6_кВ"/LConn3 -- bus15/LConn1
  _CN_160499737_110000_CN_135051666_110000/RConn1 -- "T_135051666_110000;10000;6000_ПС_53_\"Псков\"_330_110_10_6_кВ"/LConn1 -- _CN_135051666_110000_CN_175716081_110000/LConn1 -- _CN_126871068_110000_CN_135051666_110000/LConn1 -- _CN_135051666_110000_CN_202389418_110000/LConn1 -- _CN_135051666_110000_CN_250170823_110000/LConn1
  _CN_160499737_110000_CN_135051666_110000/RConn2 -- "T_135051666_110000;10000;6000_ПС_53_\"Псков\"_330_110_10_6_кВ"/LConn2 -- _CN_135051666_110000_CN_175716081_110000/LConn2 -- _CN_126871068_110000_CN_135051666_110000/LConn2 -- _CN_135051666_110000_CN_202389418_110000/LConn2 -- _CN_135051666_110000_CN_250170823_110000/LConn2
  _CN_160499737_110000_CN_135051666_110000/RConn3 -- "T_135051666_110000;10000;6000_ПС_53_\"Псков\"_330_110_10_6_кВ"/LConn3 -- _CN_135051666_110000_CN_175716081_110000/LConn3 -- bus16/LConn1 -- _CN_126871068_110000_CN_135051666_110000/LConn3 -- _CN_135051666_110000_CN_202389418_110000/LConn3 -- _CN_135051666_110000_CN_250170823_110000/LConn3
  "T_201631424_110000_ПС_126_\"Речная\"_110_6_кВ"/LConn1 -- _CN_160499737_110000_CN_201631424_110000/RConn1
  "T_201631424_110000_ПС_126_\"Речная\"_110_6_кВ"/LConn2 -- _CN_160499737_110000_CN_201631424_110000/RConn2
  _CN_160499737_110000_CN_201631424_110000/RConn3 -- "T_201631424_110000_ПС_126_\"Речная\"_110_6_кВ"/LConn3 -- bus17/LConn1
  _CN_126871068_110000_CN_135051666_110000/RConn1 -- "T_126871068_110000;6000_ПС_73_\"Льнокомбинат\"_110_6_кВ"/LConn1 -- _CN_126871068_110000_CN_116910409_110000/LConn1 -- _CN_126871068_110000_CN_202300588_110000/LConn1
  _CN_126871068_110000_CN_135051666_110000/RConn2 -- "T_126871068_110000;6000_ПС_73_\"Льнокомбинат\"_110_6_кВ"/LConn2 -- _CN_126871068_110000_CN_116910409_110000/LConn2 -- _CN_126871068_110000_CN_202300588_110000/LConn2
  _CN_126871068_110000_CN_135051666_110000/RConn3 -- "T_126871068_110000;6000_ПС_73_\"Льнокомбинат\"_110_6_кВ"/LConn3 -- _CN_126871068_110000_CN_116910409_110000/LConn3 -- _CN_126871068_110000_CN_202300588_110000/LConn3 -- bus18/LConn1
  _CN_126871068_110000_CN_116910409_110000/RConn1 -- "T_116910409_110000;10000_ПС_283_\"Завеличье\"_110_10_кВ"/LConn1 -- _CN_205085439_110000_CN_116910409_110000/LConn1
  _CN_126871068_110000_CN_116910409_110000/RConn2 -- "T_116910409_110000;10000_ПС_283_\"Завеличье\"_110_10_кВ"/LConn2 -- _CN_205085439_110000_CN_116910409_110000/LConn2
  _CN_126871068_110000_CN_116910409_110000/RConn3 -- "T_116910409_110000;10000_ПС_283_\"Завеличье\"_110_10_кВ"/LConn3 -- _CN_205085439_110000_CN_116910409_110000/LConn3 -- bus19/LConn1
  T_202300588_110000_/LConn1 -- _CN_126871068_110000_CN_202300588_110000/RConn1
  T_202300588_110000_/LConn2 -- _CN_126871068_110000_CN_202300588_110000/RConn2
  _CN_126871068_110000_CN_202300588_110000/RConn3 -- T_202300588_110000_/LConn3 -- bus20/LConn1
  _CN_175342119_110000_CN_125089960_110000/LConn1 -- "T_175342119__Подстанция_\"Невская_Дубровка\""/LConn1 -- _CN_175342119_110000_CN_175342124_110000/LConn1 -- _CN_175342119_110000_CN_160143087_110000/LConn1
  _CN_175342119_110000_CN_125089960_110000/LConn2 -- "T_175342119__Подстанция_\"Невская_Дубровка\""/LConn2 -- _CN_175342119_110000_CN_175342124_110000/LConn2 -- _CN_175342119_110000_CN_160143087_110000/LConn2
  _CN_175342119_110000_CN_125089960_110000/LConn3 -- "T_175342119__Подстанция_\"Невская_Дубровка\""/LConn3 -- _CN_175342119_110000_CN_175342124_110000/LConn3 -- _CN_175342119_110000_CN_160143087_110000/LConn3 -- bus21/LConn1
  T_125089960__ПС_382_«Кировский_ЖБИ»/LConn1 -- _CN_175342119_110000_CN_125089960_110000/RConn1
  T_125089960__ПС_382_«Кировский_ЖБИ»/LConn2 -- _CN_175342119_110000_CN_125089960_110000/RConn2
  _CN_175342119_110000_CN_125089960_110000/RConn3 -- T_125089960__ПС_382_«Кировский_ЖБИ»/LConn3 -- bus22/LConn1
  T_175342124__ПС_543_«Насосная»/LConn1 -- _CN_175342119_110000_CN_175342124_110000/RConn1
  T_175342124__ПС_543_«Насосная»/LConn2 -- _CN_175342119_110000_CN_175342124_110000/RConn2
  _CN_175342119_110000_CN_175342124_110000/RConn3 -- T_175342124__ПС_543_«Насосная»/LConn3 -- bus23/LConn1
  T_160143087__ПС_555_«Невская»/LConn1 -- _CN_175342119_110000_CN_160143087_110000/RConn1
  T_160143087__ПС_555_«Невская»/LConn2 -- _CN_175342119_110000_CN_160143087_110000/RConn2
  _CN_175342119_110000_CN_160143087_110000/RConn3 -- T_160143087__ПС_555_«Невская»/LConn3 -- bus24/LConn1
  _CN_137274923_110000_CN_79549681_110000/LConn1 -- "T_137274923__Подстанция_\"Парголово_Парнас\""/LConn1 -- _CN_137274923_110000_CN_108793849_110000/LConn1
  _CN_137274923_110000_CN_79549681_110000/LConn2 -- "T_137274923__Подстанция_\"Парголово_Парнас\""/LConn2 -- _CN_137274923_110000_CN_108793849_110000/LConn2
  _CN_137274923_110000_CN_79549681_110000/LConn3 -- "T_137274923__Подстанция_\"Парголово_Парнас\""/LConn3 -- _CN_137274923_110000_CN_108793849_110000/LConn3 -- bus25/LConn1
  "T_79549681__Подстанция_\"Прядильно_ткацкая_фабрика\""/LConn1 -- _CN_137274923_110000_CN_79549681_110000/RConn1
  "T_79549681__Подстанция_\"Прядильно_ткацкая_фабрика\""/LConn2 -- _CN_137274923_110000_CN_79549681_110000/RConn2
  _CN_137274923_110000_CN_79549681_110000/RConn3 -- "T_79549681__Подстанция_\"Прядильно_ткацкая_фабрика\""/LConn3 -- bus26/LConn1
  "T_108793849__Подстанция_\"Адамант\""/LConn1 -- _CN_137274923_110000_CN_108793849_110000/RConn1
  "T_108793849__Подстанция_\"Адамант\""/LConn2 -- _CN_137274923_110000_CN_108793849_110000/RConn2
  _CN_137274923_110000_CN_108793849_110000/RConn3 -- "T_108793849__Подстанция_\"Адамант\""/LConn3 -- bus27/LConn1
  "T_74142253__Подстанция_\"Сосновская\""/LConn1 -- _CN_74142253_110000_CN_104487370_110000/LConn1
  "T_74142253__Подстанция_\"Сосновская\""/LConn2 -- _CN_74142253_110000_CN_104487370_110000/LConn2
  _CN_74142253_110000_CN_104487370_110000/LConn3 -- "T_74142253__Подстанция_\"Сосновская\""/LConn3 -- bus28/LConn1
  "T_104487370__Подстация_\"Гражданская\""/LConn1 -- _CN_74142253_110000_CN_104487370_110000/RConn1
  "T_104487370__Подстация_\"Гражданская\""/LConn2 -- _CN_74142253_110000_CN_104487370_110000/RConn2
  _CN_74142253_110000_CN_104487370_110000/RConn3 -- "T_104487370__Подстация_\"Гражданская\""/LConn3 -- bus29/LConn1
  _CN_25913909_110000_CN_142029975_110000/LConn1 -- "T_25913909_330000_Подстанция_\"Восточная\""/RConn1 -- _CN_25913909_110000_CN_25452223_110000/LConn1 -- _CN_25913909_110000_CN_142008798_110000/LConn1 -- _CN_25913909_110000_CN_157742506_110000/LConn1 -- L_25913909/LConn1
  _CN_25913909_110000_CN_142029975_110000/LConn2 -- "T_25913909_330000_Подстанция_\"Восточная\""/RConn2 -- _CN_25913909_110000_CN_25452223_110000/LConn2 -- _CN_25913909_110000_CN_142008798_110000/LConn2 -- _CN_25913909_110000_CN_157742506_110000/LConn2 -- L_25913909/LConn2
  _CN_25913909_110000_CN_142029975_110000/LConn3 -- "T_25913909_330000_Подстанция_\"Восточная\""/RConn3 -- _CN_25913909_110000_CN_25452223_110000/LConn3 -- _CN_25913909_110000_CN_142008798_110000/LConn3 -- _CN_25913909_110000_CN_157742506_110000/LConn3 -- L_25913909/LConn3 -- bus30/LConn1
  T_142029975__ПС_№294_«Колтуши»/LConn1 -- _CN_25913909_110000_CN_142029975_110000/RConn1
  T_142029975__ПС_№294_«Колтуши»/LConn2 -- _CN_25913909_110000_CN_142029975_110000/RConn2
  _CN_25913909_110000_CN_142029975_110000/RConn3 -- T_142029975__ПС_№294_«Колтуши»/LConn3 -- bus31/LConn1
  T_25452223__ПС_525_«Ильинка»/LConn1 -- _CN_25913909_110000_CN_25452223_110000/RConn1
  T_25452223__ПС_525_«Ильинка»/LConn2 -- _CN_25913909_110000_CN_25452223_110000/RConn2
  _CN_25913909_110000_CN_25452223_110000/RConn3 -- T_25452223__ПС_525_«Ильинка»/LConn3 -- bus32/LConn1
  _CN_25913909_110000_CN_142008798_110000/RConn1 -- "T_142008798_110000_Трансформаторная_подстанция_\"Манушкино\""/LConn1 -- _CN_56029959_110000_CN_142008798_110000/LConn1
  _CN_25913909_110000_CN_142008798_110000/RConn2 -- "T_142008798_110000_Трансформаторная_подстанция_\"Манушкино\""/LConn2 -- _CN_56029959_110000_CN_142008798_110000/LConn2
  _CN_25913909_110000_CN_142008798_110000/RConn3 -- "T_142008798_110000_Трансформаторная_подстанция_\"Манушкино\""/LConn3 -- _CN_56029959_110000_CN_142008798_110000/LConn3 -- bus33/LConn1
  "T_157742506__Подстанция_\"Янино\""/LConn1 -- _CN_25913909_110000_CN_157742506_110000/RConn1
  "T_157742506__Подстанция_\"Янино\""/LConn2 -- _CN_25913909_110000_CN_157742506_110000/RConn2
  _CN_25913909_110000_CN_157742506_110000/RConn3 -- "T_157742506__Подстанция_\"Янино\""/LConn3 -- bus34/LConn1
  T_191152697__/LConn1 -- _CN_191152697_110000_CN_191545113_110000/LConn1
  T_191152697__/LConn2 -- _CN_191152697_110000_CN_191545113_110000/LConn2
  _CN_191152697_110000_CN_191545113_110000/LConn3 -- T_191152697__/LConn3 -- bus35/LConn1
  T_191545113__/LConn1 -- _CN_191152697_110000_CN_191545113_110000/RConn1
  T_191545113__/LConn2 -- _CN_191152697_110000_CN_191545113_110000/RConn2
  _CN_191152697_110000_CN_191545113_110000/RConn3 -- T_191545113__/LConn3 -- bus36/LConn1
  T_191152700__/LConn1 -- _CN_191152700_110000_CN_191054670_110000/LConn1
  T_191152700__/LConn2 -- _CN_191152700_110000_CN_191054670_110000/LConn2
  _CN_191152700_110000_CN_191054670_110000/LConn3 -- T_191152700__/LConn3 -- bus37/LConn1
  T_191054670__/LConn1 -- _CN_191152700_110000_CN_191054670_110000/RConn1
  T_191054670__/LConn2 -- _CN_191152700_110000_CN_191054670_110000/RConn2
  _CN_191152700_110000_CN_191054670_110000/RConn3 -- T_191054670__/LConn3 -- bus38/LConn1
  T_190857322__/LConn1 -- _CN_190857322_110000_CN_188266306_110000/LConn1
  T_190857322__/LConn2 -- _CN_190857322_110000_CN_188266306_110000/LConn2
  _CN_190857322_110000_CN_188266306_110000/LConn3 -- T_190857322__/LConn3 -- bus39/LConn1
  T_188266306__/LConn1 -- _CN_190857322_110000_CN_188266306_110000/RConn1
  T_188266306__/LConn2 -- _CN_190857322_110000_CN_188266306_110000/RConn2
  _CN_190857322_110000_CN_188266306_110000/RConn3 -- T_188266306__/LConn3 -- bus40/LConn1
  _CN_278548092_110000_CN_278548104_110000/LConn1 -- T_278548092__/LConn1 -- _CN_278548092_110000_CN_114922658_110000/LConn1
  _CN_278548092_110000_CN_278548104_110000/LConn2 -- T_278548092__/LConn2 -- _CN_278548092_110000_CN_114922658_110000/LConn2
  _CN_278548092_110000_CN_278548104_110000/LConn3 -- T_278548092__/LConn3 -- _CN_278548092_110000_CN_114922658_110000/LConn3 -- bus41/LConn1
  T_278548104__/LConn1 -- _CN_278548092_110000_CN_278548104_110000/RConn1
  T_278548104__/LConn2 -- _CN_278548092_110000_CN_278548104_110000/RConn2
  _CN_278548092_110000_CN_278548104_110000/RConn3 -- T_278548104__/LConn3 -- bus42/LConn1
  T_114922658_110000;35000;15000_/LConn1 -- _CN_278548092_110000_CN_114922658_110000/RConn1
  T_114922658_110000;35000;15000_/LConn2 -- _CN_278548092_110000_CN_114922658_110000/RConn2
  _CN_278548092_110000_CN_114922658_110000/RConn3 -- T_114922658_110000;35000;15000_/LConn3 -- bus43/LConn1
  "T_162782315_110000;10000_ПС_110_10_№_66_\"Ломоносовская\""/LConn1 -- _CN_162782315_110000_CN_165256814_110000/LConn1
  "T_162782315_110000;10000_ПС_110_10_№_66_\"Ломоносовская\""/LConn2 -- _CN_162782315_110000_CN_165256814_110000/LConn2
  _CN_162782315_110000_CN_165256814_110000/LConn3 -- "T_162782315_110000;10000_ПС_110_10_№_66_\"Ломоносовская\""/LConn3 -- bus44/LConn1
  T_165256814_110000;35000;10000_ПС_70_110_35_10_Жаровиха/LConn1 -- _CN_162782315_110000_CN_165256814_110000/RConn1
  T_165256814_110000;35000;10000_ПС_70_110_35_10_Жаровиха/LConn2 -- _CN_162782315_110000_CN_165256814_110000/RConn2
  _CN_162782315_110000_CN_165256814_110000/RConn3 -- T_165256814_110000;35000;10000_ПС_70_110_35_10_Жаровиха/LConn3 -- bus45/LConn1
  _CN_345141892_110000_CN_46035010_110000/LConn1 -- T_345141892__/LConn1 -- _CN_345141892_110000_CN_161733477_110000/LConn1
  _CN_345141892_110000_CN_46035010_110000/LConn2 -- T_345141892__/LConn2 -- _CN_345141892_110000_CN_161733477_110000/LConn2
  _CN_345141892_110000_CN_46035010_110000/LConn3 -- T_345141892__/LConn3 -- _CN_345141892_110000_CN_161733477_110000/LConn3 -- bus46/LConn1
  _CN_345141892_110000_CN_46035010_110000/RConn1 -- "T_46035010_220000_Подстанция_\"Колпинская\""/LConn1 -- _CN_161733477_110000_CN_46035010_110000/LConn1 -- _CN_75305342_110000_CN_46035010_110000/LConn1
  _CN_345141892_110000_CN_46035010_110000/RConn2 -- "T_46035010_220000_Подстанция_\"Колпинская\""/LConn2 -- _CN_161733477_110000_CN_46035010_110000/LConn2 -- _CN_75305342_110000_CN_46035010_110000/LConn2
  _CN_345141892_110000_CN_46035010_110000/RConn3 -- "T_46035010_220000_Подстанция_\"Колпинская\""/LConn3 -- _CN_161733477_110000_CN_46035010_110000/LConn3 -- _CN_75305342_110000_CN_46035010_110000/LConn3 -- bus47/LConn1
  _CN_345141892_110000_CN_161733477_110000/RConn1 -- "T_161733477_330000_Подстанция_\"Колпино\""/RConn1 -- _CN_161733477_110000_CN_155145070_110000/LConn1 -- _CN_161733477_110000_CN_46035010_110000/RConn1 -- _CN_161733477_110000_CN_289656575_110000/LConn1 -- _CN_161733477_110000_CN_181286875_110000/LConn1 -- L_161733477/LConn1
  _CN_345141892_110000_CN_161733477_110000/RConn2 -- "T_161733477_330000_Подстанция_\"Колпино\""/RConn2 -- _CN_161733477_110000_CN_155145070_110000/LConn2 -- _CN_161733477_110000_CN_46035010_110000/RConn2 -- _CN_161733477_110000_CN_289656575_110000/LConn2 -- _CN_161733477_110000_CN_181286875_110000/LConn2 -- L_161733477/LConn2
  _CN_345141892_110000_CN_161733477_110000/RConn3 -- "T_161733477_330000_Подстанция_\"Колпино\""/RConn3 -- _CN_161733477_110000_CN_155145070_110000/LConn3 -- _CN_161733477_110000_CN_46035010_110000/RConn3 -- _CN_161733477_110000_CN_289656575_110000/LConn3 -- _CN_161733477_110000_CN_181286875_110000/LConn3 -- L_161733477/LConn3 -- bus48/LConn1
  T_126367371__/LConn1 -- _CN_126367371_110000_CN_230114987_110000/LConn1
  T_126367371__/LConn2 -- _CN_126367371_110000_CN_230114987_110000/LConn2
  _CN_126367371_110000_CN_230114987_110000/LConn3 -- T_126367371__/LConn3 -- bus49/LConn1
  T_230114987__ЭПС/LConn1 -- _CN_126367371_110000_CN_230114987_110000/RConn1
  T_230114987__ЭПС/LConn2 -- _CN_126367371_110000_CN_230114987_110000/RConn2
  _CN_126367371_110000_CN_230114987_110000/RConn3 -- T_230114987__ЭПС/LConn3 -- bus50/LConn1
  T_206137484__ПС_43_«Гарболово»/LConn1 -- _CN_206137484_110000_CN_205542778_110000/LConn1
  T_206137484__ПС_43_«Гарболово»/LConn2 -- _CN_206137484_110000_CN_205542778_110000/LConn2
  _CN_206137484_110000_CN_205542778_110000/LConn3 -- T_206137484__ПС_43_«Гарболово»/LConn3 -- bus51/LConn1
  T_205542778__ПС_47_«Лехтуси»/LConn1 -- _CN_206137484_110000_CN_205542778_110000/RConn1
  T_205542778__ПС_47_«Лехтуси»/LConn2 -- _CN_206137484_110000_CN_205542778_110000/RConn2
  _CN_206137484_110000_CN_205542778_110000/RConn3 -- T_205542778__ПС_47_«Лехтуси»/LConn3 -- bus52/LConn1
  T_125115540_110000_/LConn1 -- _CN_125115540_110000_CN_174003451_110000/LConn1
  T_125115540_110000_/LConn2 -- _CN_125115540_110000_CN_174003451_110000/LConn2
  _CN_125115540_110000_CN_174003451_110000/LConn3 -- T_125115540_110000_/LConn3 -- bus53/LConn1
  _CN_125115540_110000_CN_174003451_110000/RConn1 -- T_174003451__ПС_515_«ГПП_2»/LConn1 -- _CN_174003451_110000_CN_152849205_110000/LConn1 -- _CN_174003451_110000_CN_179043147_110000/LConn1
  _CN_125115540_110000_CN_174003451_110000/RConn2 -- T_174003451__ПС_515_«ГПП_2»/LConn2 -- _CN_174003451_110000_CN_152849205_110000/LConn2 -- _CN_174003451_110000_CN_179043147_110000/LConn2
  _CN_125115540_110000_CN_174003451_110000/RConn3 -- T_174003451__ПС_515_«ГПП_2»/LConn3 -- _CN_174003451_110000_CN_152849205_110000/LConn3 -- _CN_174003451_110000_CN_179043147_110000/LConn3 -- bus54/LConn1
  T_153756310_110000;fixme_/LConn1 -- _CN_153756310_110000_CN_179107625_110000/LConn1
  T_153756310_110000;fixme_/LConn2 -- _CN_153756310_110000_CN_179107625_110000/LConn2
  _CN_153756310_110000_CN_179107625_110000/LConn3 -- T_153756310_110000;fixme_/LConn3 -- bus55/LConn1
  T_179107625__/LConn1 -- _CN_153756310_110000_CN_179107625_110000/RConn1
  T_179107625__/LConn2 -- _CN_153756310_110000_CN_179107625_110000/RConn2
  _CN_153756310_110000_CN_179107625_110000/RConn3 -- T_179107625__/LConn3 -- bus56/LConn1
  "T_27190951__ЭПС_\"Районная\""/LConn1 -- _CN_27190951_110000_CN_356503018_110000/LConn1
  "T_27190951__ЭПС_\"Районная\""/LConn2 -- _CN_27190951_110000_CN_356503018_110000/LConn2
  _CN_27190951_110000_CN_356503018_110000/LConn3 -- "T_27190951__ЭПС_\"Районная\""/LConn3 -- bus57/LConn1
  T_356503018__/LConn1 -- _CN_27190951_110000_CN_356503018_110000/RConn1
  T_356503018__/LConn2 -- _CN_27190951_110000_CN_356503018_110000/RConn2
  _CN_27190951_110000_CN_356503018_110000/RConn3 -- T_356503018__/LConn3 -- bus58/LConn1
  T_203028168_110000;fixme_/LConn1 -- _CN_203028168_110000_CN_203028169_110000/LConn1
  T_203028168_110000;fixme_/LConn2 -- _CN_203028168_110000_CN_203028169_110000/LConn2
  _CN_203028168_110000_CN_203028169_110000/LConn3 -- T_203028168_110000;fixme_/LConn3 -- bus59/LConn1
  _CN_203028168_110000_CN_203028169_110000/RConn1 -- T_203028169_110000;fixme_/LConn1 -- _CN_203028169_110000_CN_304918139_110000/LConn1 -- _CN_203028169_110000_CN_152869732_110000/LConn1
  _CN_203028168_110000_CN_203028169_110000/RConn2 -- T_203028169_110000;fixme_/LConn2 -- _CN_203028169_110000_CN_304918139_110000/LConn2 -- _CN_203028169_110000_CN_152869732_110000/LConn2
  _CN_203028168_110000_CN_203028169_110000/RConn3 -- T_203028169_110000;fixme_/LConn3 -- _CN_203028169_110000_CN_304918139_110000/LConn3 -- _CN_203028169_110000_CN_152869732_110000/LConn3 -- bus60/LConn1
  T_304918139_110000;35000;fixme_/LConn1 -- _CN_203028169_110000_CN_304918139_110000/RConn1
  T_304918139_110000;35000;fixme_/LConn2 -- _CN_203028169_110000_CN_304918139_110000/RConn2
  _CN_203028169_110000_CN_304918139_110000/RConn3 -- T_304918139_110000;35000;fixme_/LConn3 -- bus61/LConn1
  T_152869732__Т_П_343_11/LConn1 -- _CN_203028169_110000_CN_152869732_110000/RConn1
  T_152869732__Т_П_343_11/LConn2 -- _CN_203028169_110000_CN_152869732_110000/RConn2
  _CN_203028169_110000_CN_152869732_110000/RConn3 -- T_152869732__Т_П_343_11/LConn3 -- bus62/LConn1
  _CN_34682059_110000_CN_34682060_110000/LConn1 -- T_34682059_330000;110000_Balti_EJ_alajaam/RConn1 -- Balti_EJ_—_Narva_HEJ_110_kV_CN_34682059_110000_CN_321829090_110000/LConn1 -- _CN_34682059_110000_CN_35594708_110000/LConn1 -- _CN_34682059_110000_CN_94121285_110000/LConn1 -- L_34682059/LConn1
  _CN_34682059_110000_CN_34682060_110000/LConn2 -- T_34682059_330000;110000_Balti_EJ_alajaam/RConn2 -- Balti_EJ_—_Narva_HEJ_110_kV_CN_34682059_110000_CN_321829090_110000/LConn2 -- _CN_34682059_110000_CN_35594708_110000/LConn2 -- _CN_34682059_110000_CN_94121285_110000/LConn2 -- L_34682059/LConn2
  _CN_34682059_110000_CN_34682060_110000/LConn3 -- T_34682059_330000;110000_Balti_EJ_alajaam/RConn3 -- Balti_EJ_—_Narva_HEJ_110_kV_CN_34682059_110000_CN_321829090_110000/LConn3 -- _CN_34682059_110000_CN_35594708_110000/LConn3 -- _CN_34682059_110000_CN_94121285_110000/LConn3 -- L_34682059/LConn3 -- bus63/LConn1
  _CN_34682059_110000_CN_34682060_110000/RConn1 -- G_34682060_Balti_Elektrijaam/RConn1 -- _CN_34682059_330000_CN_34682060_110000/LConn1
  _CN_34682059_110000_CN_34682060_110000/RConn2 -- G_34682060_Balti_Elektrijaam/RConn2 -- _CN_34682059_330000_CN_34682060_110000/LConn2
  _CN_34682059_110000_CN_34682060_110000/RConn3 -- G_34682060_Balti_Elektrijaam/RConn3 -- _CN_34682059_330000_CN_34682060_110000/LConn3 -- bus64/LConn1
  T_321829090_110000;10000_Joala_alajaam/LConn1 -- Balti_EJ_—_Narva_HEJ_110_kV_CN_34682059_110000_CN_321829090_110000/RConn1
  T_321829090_110000;10000_Joala_alajaam/LConn2 -- Balti_EJ_—_Narva_HEJ_110_kV_CN_34682059_110000_CN_321829090_110000/RConn2
  Balti_EJ_—_Narva_HEJ_110_kV_CN_34682059_110000_CN_321829090_110000/RConn3 -- T_321829090_110000;10000_Joala_alajaam/LConn3 -- bus65/LConn1
  T_35594708_110000;35000;6000_Narva_Peaalajaam/LConn1 -- _CN_34682059_110000_CN_35594708_110000/RConn1
  T_35594708_110000;35000;6000_Narva_Peaalajaam/LConn2 -- _CN_34682059_110000_CN_35594708_110000/RConn2
  _CN_34682059_110000_CN_35594708_110000/RConn3 -- T_35594708_110000;35000;6000_Narva_Peaalajaam/LConn3 -- bus66/LConn1
  T_94121285_110000_Kreenholmi_alajaam/LConn1 -- _CN_34682059_110000_CN_94121285_110000/RConn1
  T_94121285_110000_Kreenholmi_alajaam/LConn2 -- _CN_34682059_110000_CN_94121285_110000/RConn2
  _CN_34682059_110000_CN_94121285_110000/RConn3 -- T_94121285_110000_Kreenholmi_alajaam/LConn3 -- bus67/LConn1
  T_162207454__/LConn1 -- _CN_162207454_110000_CN_125387022_110000/LConn1
  T_162207454__/LConn2 -- _CN_162207454_110000_CN_125387022_110000/LConn2
  _CN_162207454_110000_CN_125387022_110000/LConn3 -- T_162207454__/LConn3 -- bus68/LConn1
  T_125387022__/LConn1 -- _CN_162207454_110000_CN_125387022_110000/RConn1
  T_125387022__/LConn2 -- _CN_162207454_110000_CN_125387022_110000/RConn2
  _CN_162207454_110000_CN_125387022_110000/RConn3 -- T_125387022__/LConn3 -- bus69/LConn1
  _CN_302938336_110000_CN_73882606_110000/LConn1 -- T_302938336_330000;110000;15000_ПС_О_1_«Центральная»/RConn1 -- L_302938336/LConn1
  _CN_302938336_110000_CN_73882606_110000/LConn2 -- T_302938336_330000;110000;15000_ПС_О_1_«Центральная»/RConn2 -- L_302938336/LConn2
  _CN_302938336_110000_CN_73882606_110000/LConn3 -- T_302938336_330000;110000;15000_ПС_О_1_«Центральная»/RConn3 -- L_302938336/LConn3 -- bus70/LConn1
  T_73882606__/LConn1 -- _CN_302938336_110000_CN_73882606_110000/RConn1
  T_73882606__/LConn2 -- _CN_302938336_110000_CN_73882606_110000/RConn2
  _CN_302938336_110000_CN_73882606_110000/RConn3 -- T_73882606__/LConn3 -- bus71/LConn1
  _CN_55263465_110000_CN_165278014_110000/LConn1 -- T_55263465__Подстанция_№39/LConn1 -- _CN_55263465_110000_CN_95386425_110000/LConn1
  _CN_55263465_110000_CN_165278014_110000/LConn2 -- T_55263465__Подстанция_№39/LConn2 -- _CN_55263465_110000_CN_95386425_110000/LConn2
  _CN_55263465_110000_CN_165278014_110000/LConn3 -- T_55263465__Подстанция_№39/LConn3 -- _CN_55263465_110000_CN_95386425_110000/LConn3 -- bus72/LConn1
  T_165278014__/LConn1 -- _CN_55263465_110000_CN_165278014_110000/RConn1
  T_165278014__/LConn2 -- _CN_55263465_110000_CN_165278014_110000/RConn2
  _CN_55263465_110000_CN_165278014_110000/RConn3 -- T_165278014__/LConn3 -- bus73/LConn1
  T_95386425__ПС_№502_«Мартышкино»/LConn1 -- _CN_55263465_110000_CN_95386425_110000/RConn1
  T_95386425__ПС_№502_«Мартышкино»/LConn2 -- _CN_55263465_110000_CN_95386425_110000/RConn2
  _CN_55263465_110000_CN_95386425_110000/RConn3 -- T_95386425__ПС_№502_«Мартышкино»/LConn3 -- bus74/LConn1
  _CN_53126382_110000_CN_95829467_110000/LConn1 -- T_53126382_330000;110000;15000_ПС_«Северная_330»/RConn1 -- L_53126382/LConn1
  _CN_53126382_110000_CN_95829467_110000/LConn2 -- T_53126382_330000;110000;15000_ПС_«Северная_330»/RConn2 -- L_53126382/LConn2
  _CN_53126382_110000_CN_95829467_110000/LConn3 -- T_53126382_330000;110000;15000_ПС_«Северная_330»/RConn3 -- L_53126382/LConn3 -- bus75/LConn1
  T_95829467__Северная/LConn1 -- _CN_53126382_110000_CN_95829467_110000/RConn1
  T_95829467__Северная/LConn2 -- _CN_53126382_110000_CN_95829467_110000/RConn2
  _CN_53126382_110000_CN_95829467_110000/RConn3 -- T_95829467__Северная/LConn3 -- bus76/LConn1
  T_152849205__ПС_403_«Мельничный_Ручей»/LConn1 -- _CN_174003451_110000_CN_152849205_110000/RConn1
  T_152849205__ПС_403_«Мельничный_Ручей»/LConn2 -- _CN_174003451_110000_CN_152849205_110000/RConn2
  _CN_174003451_110000_CN_152849205_110000/RConn3 -- T_152849205__ПС_403_«Мельничный_Ручей»/LConn3 -- bus77/LConn1
  T_179043147__ПС_325_«Лепсари»/LConn1 -- _CN_174003451_110000_CN_179043147_110000/RConn1
  T_179043147__ПС_325_«Лепсари»/LConn2 -- _CN_174003451_110000_CN_179043147_110000/RConn2
  _CN_174003451_110000_CN_179043147_110000/RConn3 -- T_179043147__ПС_325_«Лепсари»/LConn3 -- bus78/LConn1
  _CN_24004349_110000_CN_24004345_110000/LConn1 -- "T_24004349_330000;110000;fixme_Подстанция_\"Северная\""/RConn1 -- L_24004349/LConn1
  _CN_24004349_110000_CN_24004345_110000/LConn2 -- "T_24004349_330000;110000;fixme_Подстанция_\"Северная\""/RConn2 -- L_24004349/LConn2
  _CN_24004349_110000_CN_24004345_110000/LConn3 -- "T_24004349_330000;110000;fixme_Подстанция_\"Северная\""/RConn3 -- L_24004349/LConn3 -- bus79/LConn1
  G_24004345_Северо_Западная_ТЭЦ/RConn1 -- _CN_24004349_110000_CN_24004345_110000/RConn1
  G_24004345_Северо_Западная_ТЭЦ/RConn2 -- _CN_24004349_110000_CN_24004345_110000/RConn2
  _CN_24004349_110000_CN_24004345_110000/RConn3 -- G_24004345_Северо_Западная_ТЭЦ/RConn3 -- bus80/LConn1
  _CN_205085439_110000_CN_116910409_110000/RConn1 -- "T_205085439_110000;35000;10000_ПС_69_\"Изборск\"_110_35_10_кВ"/LConn1 -- _CN_205085439_110000_CN_205085437_110000/LConn1
  _CN_205085439_110000_CN_116910409_110000/RConn2 -- "T_205085439_110000;35000;10000_ПС_69_\"Изборск\"_110_35_10_кВ"/LConn2 -- _CN_205085439_110000_CN_205085437_110000/LConn2
  _CN_205085439_110000_CN_116910409_110000/RConn3 -- "T_205085439_110000;35000;10000_ПС_69_\"Изборск\"_110_35_10_кВ"/LConn3 -- _CN_205085439_110000_CN_205085437_110000/LConn3 -- bus81/LConn1
  "T_205085437_110000_ПС_253_\"Тямша\"_110_10_кВ"/LConn1 -- _CN_205085439_110000_CN_205085437_110000/RConn1
  "T_205085437_110000_ПС_253_\"Тямша\"_110_10_кВ"/LConn2 -- _CN_205085439_110000_CN_205085437_110000/RConn2
  _CN_205085439_110000_CN_205085437_110000/RConn3 -- "T_205085437_110000_ПС_253_\"Тямша\"_110_10_кВ"/LConn3 -- bus82/LConn1
  T_42675970_220000_Зашекснинская/LConn1 -- _CN_42675970_110000_CN_328547675_110000/LConn1
  T_42675970_220000_Зашекснинская/LConn2 -- _CN_42675970_110000_CN_328547675_110000/LConn2
  _CN_42675970_110000_CN_328547675_110000/LConn3 -- T_42675970_220000_Зашекснинская/LConn3 -- bus83/LConn1
  T_328547675__/LConn1 -- _CN_42675970_110000_CN_328547675_110000/RConn1
  T_328547675__/LConn2 -- _CN_42675970_110000_CN_328547675_110000/RConn2
  _CN_42675970_110000_CN_328547675_110000/RConn3 -- T_328547675__/LConn3 -- bus84/LConn1
  T_56029959__ПС_526_«Форд»/LConn1 -- _CN_56029959_110000_CN_142008798_110000/RConn1
  T_56029959__ПС_526_«Форд»/LConn2 -- _CN_56029959_110000_CN_142008798_110000/RConn2
  _CN_56029959_110000_CN_142008798_110000/RConn3 -- T_56029959__ПС_526_«Форд»/LConn3 -- bus85/LConn1
  T_97385278__/LConn1 -- _CN_97385278_110000_CN_302320627_110000/LConn1
  T_97385278__/LConn2 -- _CN_97385278_110000_CN_302320627_110000/LConn2
  _CN_97385278_110000_CN_302320627_110000/LConn3 -- T_97385278__/LConn3 -- bus86/LConn1
  _CN_97385278_110000_CN_302320627_110000/RConn1 -- T_302320627__/LConn1 -- _CN_321533904_110000_CN_302320627_110000/LConn1
  _CN_97385278_110000_CN_302320627_110000/RConn2 -- T_302320627__/LConn2 -- _CN_321533904_110000_CN_302320627_110000/LConn2
  _CN_97385278_110000_CN_302320627_110000/RConn3 -- T_302320627__/LConn3 -- _CN_321533904_110000_CN_302320627_110000/LConn3 -- bus87/LConn1
  T_155145070__/LConn1 -- _CN_161733477_110000_CN_155145070_110000/RConn1
  T_155145070__/LConn2 -- _CN_161733477_110000_CN_155145070_110000/RConn2
  _CN_161733477_110000_CN_155145070_110000/RConn3 -- T_155145070__/LConn3 -- bus88/LConn1
  T_289656575__/LConn1 -- _CN_161733477_110000_CN_289656575_110000/RConn1
  T_289656575__/LConn2 -- _CN_161733477_110000_CN_289656575_110000/RConn2
  _CN_161733477_110000_CN_289656575_110000/RConn3 -- T_289656575__/LConn3 -- bus89/LConn1
  "G_181286875_ТЭЦ_ПГУ_\"ГСР_Энерго\""/RConn1 -- _CN_161733477_110000_CN_181286875_110000/RConn1
  "G_181286875_ТЭЦ_ПГУ_\"ГСР_Энерго\""/RConn2 -- _CN_161733477_110000_CN_181286875_110000/RConn2
  _CN_161733477_110000_CN_181286875_110000/RConn3 -- "G_181286875_ТЭЦ_ПГУ_\"ГСР_Энерго\""/RConn3 -- bus90/LConn1
  T_281578348__/LConn1 -- _CN_281578348_110000_CN_321533904_110000/LConn1
  T_281578348__/LConn2 -- _CN_281578348_110000_CN_321533904_110000/LConn2
  _CN_281578348_110000_CN_321533904_110000/LConn3 -- T_281578348__/LConn3 -- bus91/LConn1
  _CN_281578348_110000_CN_321533904_110000/RConn1 -- T_321533904_110000;35000;fixme_/LConn1 -- _CN_321533904_110000_CN_302320627_110000/RConn1
  _CN_281578348_110000_CN_321533904_110000/RConn2 -- T_321533904_110000;35000;fixme_/LConn2 -- _CN_321533904_110000_CN_302320627_110000/RConn2
  _CN_281578348_110000_CN_321533904_110000/RConn3 -- T_321533904_110000;35000;fixme_/LConn3 -- _CN_321533904_110000_CN_302320627_110000/RConn3 -- bus92/LConn1
  T_75305342__/LConn1 -- _CN_75305342_110000_CN_46035010_110000/RConn1
  T_75305342__/LConn2 -- _CN_75305342_110000_CN_46035010_110000/RConn2
  _CN_75305342_110000_CN_46035010_110000/RConn3 -- T_75305342__/LConn3 -- bus93/LConn1
  _CN_191502719_110000_CN_190866905_110000/LConn1 -- T_191502719__/RConn1 -- L_191502719/LConn1
  _CN_191502719_110000_CN_190866905_110000/LConn2 -- T_191502719__/RConn2 -- L_191502719/LConn2
  _CN_191502719_110000_CN_190866905_110000/LConn3 -- T_191502719__/RConn3 -- L_191502719/LConn3 -- bus94/LConn1
  _CN_191502719_110000_CN_190866905_110000/RConn1 -- G_190866905_Псковская_ГРЭС/RConn1 -- _CN_191502719_330000_CN_190866905_110000/LConn1
  _CN_191502719_110000_CN_190866905_110000/RConn2 -- G_190866905_Псковская_ГРЭС/RConn2 -- _CN_191502719_330000_CN_190866905_110000/LConn2
  _CN_191502719_110000_CN_190866905_110000/RConn3 -- G_190866905_Псковская_ГРЭС/RConn3 -- _CN_191502719_330000_CN_190866905_110000/LConn3 -- bus95/LConn1
  "T_202389418_110000;10000_ПС_282_\"Овсище\"_110_10_кВ"/LConn1 -- _CN_135051666_110000_CN_202389418_110000/RConn1
  "T_202389418_110000;10000_ПС_282_\"Овсище\"_110_10_кВ"/LConn2 -- _CN_135051666_110000_CN_202389418_110000/RConn2
  _CN_135051666_110000_CN_202389418_110000/RConn3 -- "T_202389418_110000;10000_ПС_282_\"Овсище\"_110_10_кВ"/LConn3 -- bus96/LConn1
  T_250170823_110000_/LConn1 -- _CN_135051666_110000_CN_250170823_110000/RConn1
  T_250170823_110000_/LConn2 -- _CN_135051666_110000_CN_250170823_110000/RConn2
  _CN_135051666_110000_CN_250170823_110000/RConn3 -- T_250170823_110000_/LConn3 -- bus97/LConn1
  "T_175716081__ПС_100_\"Северная\"_110_10_кВ"/LConn1 -- _CN_135051666_110000_CN_175716081_110000/RConn1
  "T_175716081__ПС_100_\"Северная\"_110_10_кВ"/LConn2 -- _CN_135051666_110000_CN_175716081_110000/RConn2
  _CN_135051666_110000_CN_175716081_110000/RConn3 -- "T_175716081__ПС_100_\"Северная\"_110_10_кВ"/LConn3 -- bus98/LConn1
  "T_252106171__ПС_110_кВ_\"Весьегонск\""/LConn1 -- _CN_252106171_110000_CN_252345291_110000/LConn1
  "T_252106171__ПС_110_кВ_\"Весьегонск\""/LConn2 -- _CN_252106171_110000_CN_252345291_110000/LConn2
  _CN_252106171_110000_CN_252345291_110000/LConn3 -- "T_252106171__ПС_110_кВ_\"Весьегонск\""/LConn3 -- bus99/LConn1
  "T_252345291__ПС_110_кВ_\"Сандово\""/LConn1 -- _CN_252106171_110000_CN_252345291_110000/RConn1
  "T_252345291__ПС_110_кВ_\"Сандово\""/LConn2 -- _CN_252106171_110000_CN_252345291_110000/RConn2
  _CN_252106171_110000_CN_252345291_110000/RConn3 -- "T_252345291__ПС_110_кВ_\"Сандово\""/LConn3 -- bus100/LConn1
  T_279665111_110000;15000_/LConn1 -- _CN_279665111_110000_CN_84126712_110000/LConn1
  T_279665111_110000;15000_/LConn2 -- _CN_279665111_110000_CN_84126712_110000/LConn2
  _CN_279665111_110000_CN_84126712_110000/LConn3 -- T_279665111_110000;15000_/LConn3 -- bus101/LConn1
  G_84126712_Гусевская_ТЭЦ/RConn1 -- _CN_279665111_110000_CN_84126712_110000/RConn1
  G_84126712_Гусевская_ТЭЦ/RConn2 -- _CN_279665111_110000_CN_84126712_110000/RConn2
  _CN_279665111_110000_CN_84126712_110000/RConn3 -- G_84126712_Гусевская_ТЭЦ/RConn3 -- bus102/LConn1
  "T_63107712_330000_Подстанция_\"Южная\""/LConn1 -- _CN_63107712_220000_CN_30831480_220000/LConn1
  "T_63107712_330000_Подстанция_\"Южная\""/LConn2 -- _CN_63107712_220000_CN_30831480_220000/LConn2
  _CN_63107712_220000_CN_30831480_220000/LConn3 -- "T_63107712_330000_Подстанция_\"Южная\""/LConn3 -- bus103/LConn1
  G_30831480_Южная_ТЭЦ_22/RConn1 -- _CN_63107712_220000_CN_30831480_220000/RConn1
  G_30831480_Южная_ТЭЦ_22/RConn2 -- _CN_63107712_220000_CN_30831480_220000/RConn2
  _CN_63107712_220000_CN_30831480_220000/RConn3 -- G_30831480_Южная_ТЭЦ_22/RConn3 -- bus104/LConn1
  _CN_87430145_220000_CN_106941567_220000/LConn1 -- T_87430145_220000_Печора/LConn1 -- _CN_87430145_220000_CN_88433653_220000/LConn1 -- _CN_87430145_220000_CN_105528914_220000/LConn1
  _CN_87430145_220000_CN_106941567_220000/LConn2 -- T_87430145_220000_Печора/LConn2 -- _CN_87430145_220000_CN_88433653_220000/LConn2 -- _CN_87430145_220000_CN_105528914_220000/LConn2
  _CN_87430145_220000_CN_106941567_220000/LConn3 -- T_87430145_220000_Печора/LConn3 -- _CN_87430145_220000_CN_88433653_220000/LConn3 -- _CN_87430145_220000_CN_105528914_220000/LConn3 -- bus105/LConn1
  T_106941567_220000_Северная/LConn1 -- _CN_87430145_220000_CN_106941567_220000/RConn1
  T_106941567_220000_Северная/LConn2 -- _CN_87430145_220000_CN_106941567_220000/RConn2
  _CN_87430145_220000_CN_106941567_220000/RConn3 -- T_106941567_220000_Северная/LConn3 -- bus106/LConn1
  _CN_87430145_220000_CN_88433653_220000/RConn1 -- T_88433653_220000;35000;10000_Инта_220/LConn1 -- ВЛ_220_кВ_Инта___Воркута_CN_177805996_220000_CN_88433653_220000/LConn1
  _CN_87430145_220000_CN_88433653_220000/RConn2 -- T_88433653_220000;35000;10000_Инта_220/LConn2 -- ВЛ_220_кВ_Инта___Воркута_CN_177805996_220000_CN_88433653_220000/LConn2
  _CN_87430145_220000_CN_88433653_220000/RConn3 -- T_88433653_220000;35000;10000_Инта_220/LConn3 -- ВЛ_220_кВ_Инта___Воркута_CN_177805996_220000_CN_88433653_220000/LConn3 -- bus107/LConn1
  _CN_87430145_220000_CN_105528914_220000/RConn1 -- T_105528914_220000_Усинская/LConn1 -- Усинская___Промысловая_CN_105535524_220000_CN_105528914_220000/LConn1 -- _CN_260127849_220000_CN_105528914_220000/LConn1 -- Усинская___Возейская_CN_105528914_220000_CN_260124523_220000/LConn1 -- Усинская___КС_УГПЗ_CN_105528914_220000_CN_331932782_220000/LConn1
  _CN_87430145_220000_CN_105528914_220000/RConn2 -- T_105528914_220000_Усинская/LConn2 -- Усинская___Промысловая_CN_105535524_220000_CN_105528914_220000/LConn2 -- _CN_260127849_220000_CN_105528914_220000/LConn2 -- Усинская___Возейская_CN_105528914_220000_CN_260124523_220000/LConn2 -- Усинская___КС_УГПЗ_CN_105528914_220000_CN_331932782_220000/LConn2
  _CN_87430145_220000_CN_105528914_220000/RConn3 -- T_105528914_220000_Усинская/LConn3 -- Усинская___Промысловая_CN_105535524_220000_CN_105528914_220000/LConn3 -- _CN_260127849_220000_CN_105528914_220000/LConn3 -- Усинская___Возейская_CN_105528914_220000_CN_260124523_220000/LConn3 -- Усинская___КС_УГПЗ_CN_105528914_220000_CN_331932782_220000/LConn3 -- bus108/LConn1
  "T_152126979_220000_ПС_220_кВ_\"Ухта\""/LConn1 -- Ухта___Синдор_CN_152126979_220000_CN_212471066_220000/LConn1
  "T_152126979_220000_ПС_220_кВ_\"Ухта\""/LConn2 -- Ухта___Синдор_CN_152126979_220000_CN_212471066_220000/LConn2
  Ухта___Синдор_CN_152126979_220000_CN_212471066_220000/LConn3 -- "T_152126979_220000_ПС_220_кВ_\"Ухта\""/LConn3 -- bus109/LConn1
  Ухта___Синдор_CN_152126979_220000_CN_212471066_220000/RConn1 -- T_212471066_220000_Синдор/LConn1 -- Синдор___Микунь_CN_212471066_220000_CN_211036038_220000/LConn1
  Ухта___Синдор_CN_152126979_220000_CN_212471066_220000/RConn2 -- T_212471066_220000_Синдор/LConn2 -- Синдор___Микунь_CN_212471066_220000_CN_211036038_220000/LConn2
  Ухта___Синдор_CN_152126979_220000_CN_212471066_220000/RConn3 -- T_212471066_220000_Синдор/LConn3 -- Синдор___Микунь_CN_212471066_220000_CN_211036038_220000/LConn3 -- bus110/LConn1
  _CN_133263110_220000_CN_163640749_220000/LConn1 -- T_133263110_220000_Няндома/LConn1 -- _CN_133263110_220000_CN_96836497_220000/LConn1 -- _CN_133263110_220000_CN_147416198_220000/LConn1
  _CN_133263110_220000_CN_163640749_220000/LConn2 -- T_133263110_220000_Няндома/LConn2 -- _CN_133263110_220000_CN_96836497_220000/LConn2 -- _CN_133263110_220000_CN_147416198_220000/LConn2
